simulink model "RealLifeTrainModel"  (R2024a)
settings: Solver=ode1  StartTime=0.0  StopTime=Inf  FixedStep=0.001  RelTol=1e-3
PostLoadFcn:
  | , if any(exist('dsrtsu_mdlpostloadfcn', 'file') ~= 0), dsrtsu_mdlpostloadfcn('Execute', bdroot); end,
InitFcn:
  | , if any(exist('rtifpga_mdlclblib', 'file') ~= 0), rtifpga_mdlclblib('Init', bdroot); end,
undefined symbols (not defined in the file): DiscIntNeverNeededParam
libraries: deeplib x29, svdutilitieslib x28, simulink x8, eeGeneralControl x8, rti1202lib_adc_class1 x6, rti1202serlib x5, spsEdgeDetectorLib x5, rtiemclib x2, rti1202lib_dac_class1 x1
(part 1 of 8)
Description:
  | Standard RTI1202 template.
  | Supported MATLAB version:  R2024a.
settings Model: Tag=RTI1202  DSRTSU_INTERNAL_RTI_VER=640  DSRTSU_INTERNAL_RTI_TYPE=rti1202  RTICANMMDATA=struct('GeneralSetupData',struct('modelroot','C:\Users\VM-User\Desktop\MigrationScripts','generalsettings',struct('filesettings',struct('destfolder',struct('Name','RTICANMM_FILES','Check',1),'buildfolder',struct('Name','.','Check',1),'AbsDestfolder',struct('Name','C:\Users\VM-User\Desktop\MigrationScripts\RTICANMM_FILES'),'AbsBuildfolder',struct('Name','C:\Users\VM-User\Desktop\MigrationScripts'))),'options',struct('addpaths',1,'rmpaths',1,'addtrcexclusion',true,'cannavigator',struct('checkmonitoring',0),'show_usrtrc',0,'use_usrtrc',0),'advanced',struct('options',ones(1,100)),'MPSetup',{{}},'RTI',struct('Type','RTI1202','Ver','7.17','Date','02-Nov-2021'),'modelname','','block','untitled'))  DSRTSU_INTERNAL_RTIFPGA=210  DSRTSU_INTERNAL_RTISTBM_VER=24.1  Creator=ic2d  LastModifiedBy=ic2d
settings SolverCC: AlgebraicLoopSolver=TrustRegion
settings DataIOCC: ReturnWorkspaceOutputs=off
settings OptimizationCC: BlockReduction=off  OptimizeBlockIOStorage=off  BufferReuse=off  ReuseModelBlockBuffer=off  GlobalBufferReuse=off  ExpressionFolding=off  LocalBlockOutputs=off  OptimizeDataStoreBuffers=off  BusAssignmentInplaceUpdate=off
settings DebuggingCC: MultiTaskDSMMsg=none  UnconnectedInputMsg=warning  UnconnectedOutputMsg=warning  UnconnectedLineMsg=warning  PregeneratedLibrarySubsystemCodeDiagnostic=none  ForceCombineOutputUpdateInSim=on  ArithmeticOperatorsInVariantConditions=warning
settings HardwareCC: ProdBitPerPointer=32  ProdBitPerSizeT=32  ProdBitPerPtrDiffT=32  ProdLargestAtomicInteger=Integer  ProdEndianess=BigEndian  ProdWordSize=32  ProdLongLongMode=on  ProdHWDeviceType=Custom Processor->Custom  TargetIntDivRoundTo=Zero  TargetEndianess=BigEndian  TargetHWDeviceType=Custom Processor->Custom
settings ModelReferenceCC: EnableRefExpFcnMdlSchedulingChecks=on  EnableParallelModelReferenceBuilds=on  ParallelModelReferenceMATLABWorkerInit=Load Top Model
settings SFSimCC: SimUseLocalCustomCode=off  MATLABDynamicMemAlloc=off  CustomCodeUndefinedFunction=UseInterfaceOnly
settings RTWCC: Description=dSPACE DS1202 Hardware Platform  SystemTargetFile=rti1202.tlc  MakeCommand=make_rti  TemplateMakefile=rti1202.tmf  RTWUseLocalCustomCode=off  GPUComputeCapability=3.5  DLArmComputeVersion=19.05
settings CodeAppCC: StateflowObjectComments=on
settings STFCustomTargetCC: TargetLangStandard=C89/C90 (ANSI)  ParMdlRefBuildCompliant=on  GRTInterface=off  UseToolchainInfoCompliant=off  SystemTargetFile=rti1202.tlc
settings GRTTargetCC: TargetLangStandard=C89/C90 (ANSI)  CompOptLevelCompliant=off  ConcurrentExecutionCompliant=off  CombineOutputUpdateFcns=off  MatFileLogging=off  CPPClassGenCompliant=off  UseToolchainInfoCompliant=off
settings ConfigComp: CovMetricSettings=dswe

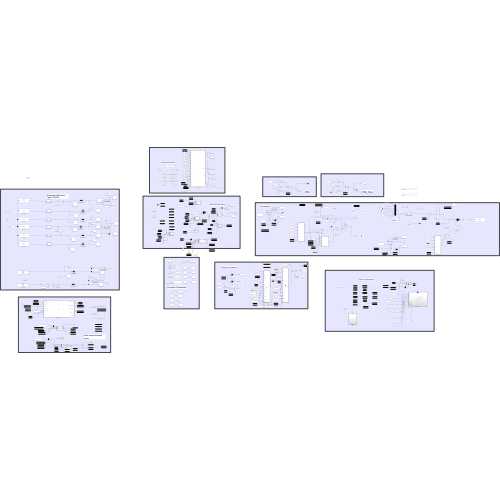
[thumbnail: Simulink's stored preview of the top-level diagram]
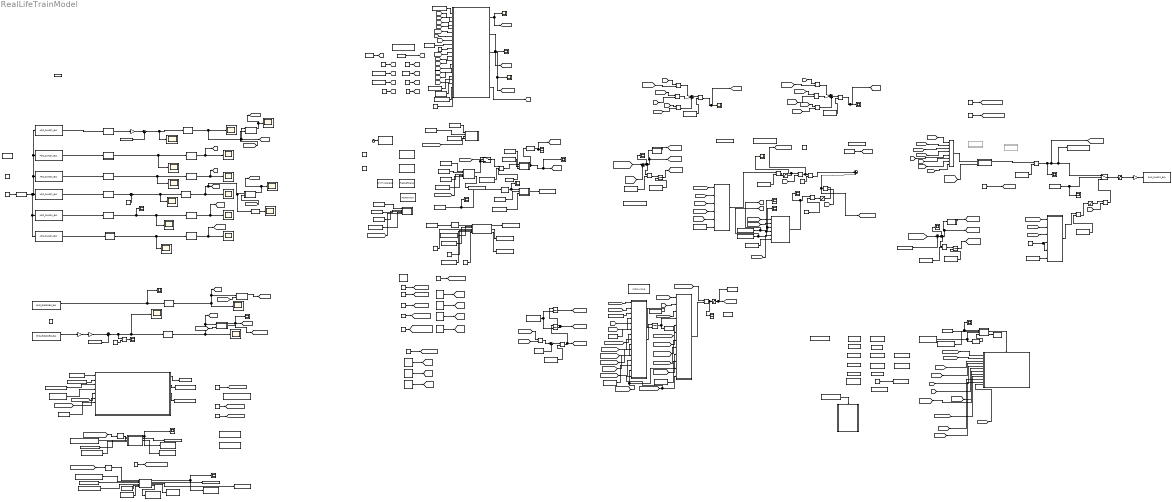
== system RealLifeTrainModel ==
  note: PID
  note: Start-Stop-Recording Logic
  note: Disturbance Estimation
  note: Controllers
  note: Hyd Model Parameters
  note: Controller Parameters
  note: Reference Generation
  note: Serial Communication
  note: Hardware Abstraction Layer (TODO)
  note: PID_Pos
  ADCReadToNewtons_Hyd : MATLAB Function  TreatAsAtomicUnit=on
  ADCReadToNewtons_Load : MATLAB Function  TreatAsAtomicUnit=on
  ADCReadToPressure : MATLAB Function  TreatAsAtomicUnit=on
  ADCReadToPressure1 : MATLAB Function  TreatAsAtomicUnit=on
  ADCReadToPressure2 : MATLAB Function  TreatAsAtomicUnit=on
  ADCReadToPressure3 : MATLAB Function  TreatAsAtomicUnit=on
  ADC_CLASS1_BL1 : rti1202lib_adc_class1/ADC_CLASS1_BL1  DSProperties=struct('RTI',struct('Version',uint32(1),'BlockType',struct('isSLSource',uint8(1),'isSLSink',uint8(1),'isHWSource',uint8(0),'isHWSink',uint8(1),'isSetup',uint8(0),'isInline',uint8(1),'isNonInline',uint8(0),'isInterrupt',uint8(0),'isChannelwise',uint8(1)),'IOBoardType',{{'DS120X','STD','ADCC1'}},'UnitType','ADC','Identifier','ADC','DialogType','ML','BlockSet','NONE','SlaveProcessor','NONE'))  RTIBlockInterface=struct('InputPortsActive',1,'InputPortsWidth',int32(1),'InputPortsDataType',{{'SS_BOOLEAN'}},'InputPortsName',{{'Continue'}},'OutputPortsActive',[1 0],'OutputPortsWidth',int32([100 1]),'OutputPortsDataType',{{'SS_DOUBLE','SS_INT16'}},'OutputPortsName',{{'ADC','Status'}},'DialogFcn','rti120xstdadcc1adcgui','SampleTime',{{-1}},'InitLevel',3,'IconTransparency','on','BlockDisplay',{{['ADC CL1\nChannel: 1'],'center'}},'BlockName',struct('Token',{{'ADC_CLASS1_BL1'}}))  RTIBlockParameters=struct('ReadMode',{{2,'OFF',[1 2]}},'ChannelNo',{{1,'OFF',[]}},'ConversionMode',{{2,'OFF',[1 2]}},'TriggerSource',{{1,'OFF',[1 2]}},'TriggerLineIn',{{1,'OFF',[1 16]}},'SampleMode',{{2,'OFF',[1 2]}},'BurstTriggerSource',{{1,'OFF',[1 2]}},'BurstTriggerLine',{{1,'OFF',[1 16]}},'ConvTriggerSource',{{3,'OFF',[1 3]}},'ConvTriggerLine',{{1,'OFF',[1 16]}},'ConvPeriod',{{'str2num(get_param(''Teste_PID/TimerValue'',''Value''))','OFF',[1e-6 1.34]}},'ConvPeriodCheck',{{1,'OFF',[]}},'BurstSize',{{'str2num(get_param(''Teste_PID/BufferSize'',''Value''))','OFF',[]}},'BurstSizeCheck',{{1,'OFF',[]}},'DataSetOffset',{{'0','OFF',[]}},'DataSetOffsetCheck',{{0,'OFF',[]}},'DataSetLength',{{'1','OFF',[]}},'DataSetLengthCheck',{{0,'OFF',[]}},'EnableTriggerEvent',{{0,'OFF',[0 1]}},'TriggerMode',{{2,'OFF',[1 3]}},'TriggerLineOut',{{1,'OFF',[1 16]}},'ADCSWStartEnable',{{0,'OFF',[0 1]}},'SampleTime',{{'-1','OFF',[-1 inf]}},'SampleTimeCheck',{{0,'OFF',[]}},'StatusPortEnable',{{0,'OFF',[0 1]}},'TLCFileName',{{'rti120xadc_c1_adc','OFF',[]}})  RTISFcnParameters=struct('ReadMode','int16','ChannelNo','int16','ConversionMode','int16','TriggerSource','int16','TriggerLineIn','int16','SampleMode','int16','BurstTriggerSource','int16','BurstTriggerLine','int16','ConvTriggerSource','int16','ConvTriggerLine','int16','ConvPeriod','double','BurstSize','int16','DataSetOffset','int16','DataSetLength','int16','EnableTriggerEvent','int16','TriggerMode','int16','TriggerLineOut','int16','ADCSWStartEnable','int16','SampleTime','double','StatusPortEnable','int16','TLCFileName','char')  RTIBlockParaDefault=struct('ReadMode',1,'ChannelNo',1,'ConversionMode',1,'TriggerSource',1,'TriggerLineIn',1,'SampleMode',1,'BurstTriggerSource',1,'BurstTriggerLine',1,'ConvTriggerSource',3,'ConvTriggerLine',1,'ConvPeriod',0.0001,'ConvPeriodCheck',0,'BurstSize',10,'BurstSizeCheck',0,'DataSetOffset',0,'DataSetOffsetCheck',0,'DataSetLength',1,'DataSetLengthCheck',0,'EnableTriggerEvent',0,'TriggerMode',2,'TriggerLineOut',1,'ADCSWStartEnable',0,'SampleTime',-1,'SampleTimeCheck',1,'StatusPortEnable',0,'TLCFileName','rti120xadc_c1_adc')
  ADC_CLASS1_BL2 : rti1202lib_adc_class1/ADC_CLASS1_BL1  DSProperties=struct('RTI',struct('Version',uint32(1),'BlockType',struct('isSLSource',uint8(1),'isSLSink',uint8(1),'isHWSource',uint8(0),'isHWSink',uint8(1),'isSetup',uint8(0),'isInline',uint8(1),'isNonInline',uint8(0),'isInterrupt',uint8(0),'isChannelwise',uint8(1)),'IOBoardType',{{'DS120X','STD','ADCC1'}},'UnitType','ADC','Identifier','ADC','DialogType','ML','BlockSet','NONE','SlaveProcessor','NONE'))  RTIBlockInterface=struct('InputPortsActive',1,'InputPortsWidth',int32(1),'InputPortsDataType',{{'SS_BOOLEAN'}},'InputPortsName',{{'Continue'}},'OutputPortsActive',[1 0],'OutputPortsWidth',int32([100 1]),'OutputPortsDataType',{{'SS_DOUBLE','SS_INT16'}},'OutputPortsName',{{'ADC','Status'}},'DialogFcn','rti120xstdadcc1adcgui','SampleTime',{{-1}},'InitLevel',3,'IconTransparency','on','BlockDisplay',{{['ADC CL1\nChannel: 13'],'center'}},'BlockName',struct('Token',{{'ADC_CLASS1_BL1'}}))  RTIBlockParameters=struct('ReadMode',{{2,'OFF',[1 2]}},'ChannelNo',{{13,'OFF',[]}},'ConversionMode',{{2,'OFF',[1 2]}},'TriggerSource',{{1,'OFF',[1 2]}},'TriggerLineIn',{{1,'OFF',[1 16]}},'SampleMode',{{2,'OFF',[1 2]}},'BurstTriggerSource',{{1,'OFF',[1 2]}},'BurstTriggerLine',{{1,'OFF',[1 16]}},'ConvTriggerSource',{{3,'OFF',[1 3]}},'ConvTriggerLine',{{1,'OFF',[1 16]}},'ConvPeriod',{{'str2num(get_param(''Teste_PID/TimerValue'',''Value''))','OFF',[1e-6 1.34]}},'ConvPeriodCheck',{{1,'OFF',[]}},'BurstSize',{{'str2num(get_param(''Teste_PID/BufferSize'',''Value''))','OFF',[]}},'BurstSizeCheck',{{1,'OFF',[]}},'DataSetOffset',{{'0','OFF',[]}},'DataSetOffsetCheck',{{0,'OFF',[]}},'DataSetLength',{{'1','OFF',[]}},'DataSetLengthCheck',{{0,'OFF',[]}},'EnableTriggerEvent',{{0,'OFF',[0 1]}},'TriggerMode',{{2,'OFF',[1 3]}},'TriggerLineOut',{{1,'OFF',[1 16]}},'ADCSWStartEnable',{{0,'OFF',[0 1]}},'SampleTime',{{'-1','OFF',[-1 inf]}},'SampleTimeCheck',{{0,'OFF',[]}},'StatusPortEnable',{{0,'OFF',[0 1]}},'TLCFileName',{{'rti120xadc_c1_adc','OFF',[]}})  RTISFcnParameters=struct('ReadMode','int16','ChannelNo','int16','ConversionMode','int16','TriggerSource','int16','TriggerLineIn','int16','SampleMode','int16','BurstTriggerSource','int16','BurstTriggerLine','int16','ConvTriggerSource','int16','ConvTriggerLine','int16','ConvPeriod','double','BurstSize','int16','DataSetOffset','int16','DataSetLength','int16','EnableTriggerEvent','int16','TriggerMode','int16','TriggerLineOut','int16','ADCSWStartEnable','int16','SampleTime','double','StatusPortEnable','int16','TLCFileName','char')  RTIBlockParaDefault=struct('ReadMode',1,'ChannelNo',1,'ConversionMode',1,'TriggerSource',1,'TriggerLineIn',1,'SampleMode',1,'BurstTriggerSource',1,'BurstTriggerLine',1,'ConvTriggerSource',3,'ConvTriggerLine',1,'ConvPeriod',0.0001,'ConvPeriodCheck',0,'BurstSize',10,'BurstSizeCheck',0,'DataSetOffset',0,'DataSetOffsetCheck',0,'DataSetLength',1,'DataSetLengthCheck',0,'EnableTriggerEvent',0,'TriggerMode',2,'TriggerLineOut',1,'ADCSWStartEnable',0,'SampleTime',-1,'SampleTimeCheck',1,'StatusPortEnable',0,'TLCFileName','rti120xadc_c1_adc')
  ADC_CLASS1_BL3 : rti1202lib_adc_class1/ADC_CLASS1_BL1  DSProperties=struct('RTI',struct('Version',uint32(1),'BlockType',struct('isSLSource',uint8(1),'isSLSink',uint8(1),'isHWSource',uint8(0),'isHWSink',uint8(1),'isSetup',uint8(0),'isInline',uint8(1),'isNonInline',uint8(0),'isInterrupt',uint8(0),'isChannelwise',uint8(1)),'IOBoardType',{{'DS120X','STD','ADCC1'}},'UnitType','ADC','Identifier','ADC','DialogType','ML','BlockSet','NONE','SlaveProcessor','NONE'))  RTIBlockInterface=struct('InputPortsActive',1,'InputPortsWidth',int32(1),'InputPortsDataType',{{'SS_BOOLEAN'}},'InputPortsName',{{'Continue'}},'OutputPortsActive',[1 0],'OutputPortsWidth',int32([100 1]),'OutputPortsDataType',{{'SS_DOUBLE','SS_INT16'}},'OutputPortsName',{{'ADC','Status'}},'DialogFcn','rti120xstdadcc1adcgui','SampleTime',{{-1}},'InitLevel',3,'IconTransparency','on','BlockDisplay',{{['ADC CL1\nChannel: 5'],'center'}},'BlockName',struct('Token',{{'ADC_CLASS1_BL1'}}))  RTIBlockParameters=struct('ReadMode',{{2,'OFF',[1 2]}},'ChannelNo',{{5,'OFF',[]}},'ConversionMode',{{2,'OFF',[1 2]}},'TriggerSource',{{1,'OFF',[1 2]}},'TriggerLineIn',{{1,'OFF',[1 16]}},'SampleMode',{{2,'OFF',[1 2]}},'BurstTriggerSource',{{1,'OFF',[1 2]}},'BurstTriggerLine',{{1,'OFF',[1 16]}},'ConvTriggerSource',{{3,'OFF',[1 3]}},'ConvTriggerLine',{{1,'OFF',[1 16]}},'ConvPeriod',{{'str2num(get_param(''Teste_PID/TimerValue'',''Value''))','OFF',[1e-6 1.34]}},'ConvPeriodCheck',{{1,'OFF',[]}},'BurstSize',{{'str2num(get_param(''Teste_PID/BufferSize'',''Value''))','OFF',[]}},'BurstSizeCheck',{{1,'OFF',[]}},'DataSetOffset',{{'0','OFF',[]}},'DataSetOffsetCheck',{{0,'OFF',[]}},'DataSetLength',{{'1','OFF',[]}},'DataSetLengthCheck',{{0,'OFF',[]}},'EnableTriggerEvent',{{0,'OFF',[0 1]}},'TriggerMode',{{2,'OFF',[1 3]}},'TriggerLineOut',{{1,'OFF',[1 16]}},'ADCSWStartEnable',{{0,'OFF',[0 1]}},'SampleTime',{{'-1','OFF',[-1 inf]}},'SampleTimeCheck',{{0,'OFF',[]}},'StatusPortEnable',{{0,'OFF',[0 1]}},'TLCFileName',{{'rti120xadc_c1_adc','OFF',[]}})  RTISFcnParameters=struct('ReadMode','int16','ChannelNo','int16','ConversionMode','int16','TriggerSource','int16','TriggerLineIn','int16','SampleMode','int16','BurstTriggerSource','int16','BurstTriggerLine','int16','ConvTriggerSource','int16','ConvTriggerLine','int16','ConvPeriod','double','BurstSize','int16','DataSetOffset','int16','DataSetLength','int16','EnableTriggerEvent','int16','TriggerMode','int16','TriggerLineOut','int16','ADCSWStartEnable','int16','SampleTime','double','StatusPortEnable','int16','TLCFileName','char')  RTIBlockParaDefault=struct('ReadMode',1,'ChannelNo',1,'ConversionMode',1,'TriggerSource',1,'TriggerLineIn',1,'SampleMode',1,'BurstTriggerSource',1,'BurstTriggerLine',1,'ConvTriggerSource',3,'ConvTriggerLine',1,'ConvPeriod',0.0001,'ConvPeriodCheck',0,'BurstSize',10,'BurstSizeCheck',0,'DataSetOffset',0,'DataSetOffsetCheck',0,'DataSetLength',1,'DataSetLengthCheck',0,'EnableTriggerEvent',0,'TriggerMode',2,'TriggerLineOut',1,'ADCSWStartEnable',0,'SampleTime',-1,'SampleTimeCheck',1,'StatusPortEnable',0,'TLCFileName','rti120xadc_c1_adc')
  ADC_CLASS1_BL4 : rti1202lib_adc_class1/ADC_CLASS1_BL1  DSProperties=struct('RTI',struct('Version',uint32(1),'BlockType',struct('isSLSource',uint8(1),'isSLSink',uint8(1),'isHWSource',uint8(0),'isHWSink',uint8(1),'isSetup',uint8(0),'isInline',uint8(1),'isNonInline',uint8(0),'isInterrupt',uint8(0),'isChannelwise',uint8(1)),'IOBoardType',{{'DS120X','STD','ADCC1'}},'UnitType','ADC','Identifier','ADC','DialogType','ML','BlockSet','NONE','SlaveProcessor','NONE'))  RTIBlockInterface=struct('InputPortsActive',1,'InputPortsWidth',int32(1),'InputPortsDataType',{{'SS_BOOLEAN'}},'InputPortsName',{{'Continue'}},'OutputPortsActive',[1 0],'OutputPortsWidth',int32([100 1]),'OutputPortsDataType',{{'SS_DOUBLE','SS_INT16'}},'OutputPortsName',{{'ADC','Status'}},'DialogFcn','rti120xstdadcc1adcgui','SampleTime',{{-1}},'InitLevel',3,'IconTransparency','on','BlockDisplay',{{['ADC CL1\nChannel: 2'],'center'}},'BlockName',struct('Token',{{'ADC_CLASS1_BL1'}}))  RTIBlockParameters=struct('ReadMode',{{2,'OFF',[1 2]}},'ChannelNo',{{2,'OFF',[]}},'ConversionMode',{{2,'OFF',[1 2]}},'TriggerSource',{{1,'OFF',[1 2]}},'TriggerLineIn',{{1,'OFF',[1 16]}},'SampleMode',{{2,'OFF',[1 2]}},'BurstTriggerSource',{{1,'OFF',[1 2]}},'BurstTriggerLine',{{1,'OFF',[1 16]}},'ConvTriggerSource',{{3,'OFF',[1 3]}},'ConvTriggerLine',{{1,'OFF',[1 16]}},'ConvPeriod',{{'str2num(get_param(''Teste_PID/TimerValue'',''Value''))','OFF',[1e-6 1.34]}},'ConvPeriodCheck',{{1,'OFF',[]}},'BurstSize',{{'str2num(get_param(''Teste_PID/BufferSize'',''Value''))','OFF',[]}},'BurstSizeCheck',{{1,'OFF',[]}},'DataSetOffset',{{'0','OFF',[]}},'DataSetOffsetCheck',{{0,'OFF',[]}},'DataSetLength',{{'1','OFF',[]}},'DataSetLengthCheck',{{0,'OFF',[]}},'EnableTriggerEvent',{{0,'OFF',[0 1]}},'TriggerMode',{{2,'OFF',[1 3]}},'TriggerLineOut',{{1,'OFF',[1 16]}},'ADCSWStartEnable',{{0,'OFF',[0 1]}},'SampleTime',{{'-1','OFF',[-1 inf]}},'SampleTimeCheck',{{0,'OFF',[]}},'StatusPortEnable',{{0,'OFF',[0 1]}},'TLCFileName',{{'rti120xadc_c1_adc','OFF',[]}})  RTISFcnParameters=struct('ReadMode','int16','ChannelNo','int16','ConversionMode','int16','TriggerSource','int16','TriggerLineIn','int16','SampleMode','int16','BurstTriggerSource','int16','BurstTriggerLine','int16','ConvTriggerSource','int16','ConvTriggerLine','int16','ConvPeriod','double','BurstSize','int16','DataSetOffset','int16','DataSetLength','int16','EnableTriggerEvent','int16','TriggerMode','int16','TriggerLineOut','int16','ADCSWStartEnable','int16','SampleTime','double','StatusPortEnable','int16','TLCFileName','char')  RTIBlockParaDefault=struct('ReadMode',1,'ChannelNo',1,'ConversionMode',1,'TriggerSource',1,'TriggerLineIn',1,'SampleMode',1,'BurstTriggerSource',1,'BurstTriggerLine',1,'ConvTriggerSource',3,'ConvTriggerLine',1,'ConvPeriod',0.0001,'ConvPeriodCheck',0,'BurstSize',10,'BurstSizeCheck',0,'DataSetOffset',0,'DataSetOffsetCheck',0,'DataSetLength',1,'DataSetLengthCheck',0,'EnableTriggerEvent',0,'TriggerMode',2,'TriggerLineOut',1,'ADCSWStartEnable',0,'SampleTime',-1,'SampleTimeCheck',1,'StatusPortEnable',0,'TLCFileName','rti120xadc_c1_adc')
  ADC_CLASS1_BL5 : rti1202lib_adc_class1/ADC_CLASS1_BL1  DSProperties=struct('RTI',struct('Version',uint32(1),'BlockType',struct('isSLSource',uint8(1),'isSLSink',uint8(1),'isHWSource',uint8(0),'isHWSink',uint8(1),'isSetup',uint8(0),'isInline',uint8(1),'isNonInline',uint8(0),'isInterrupt',uint8(0),'isChannelwise',uint8(1)),'IOBoardType',{{'DS120X','STD','ADCC1'}},'UnitType','ADC','Identifier','ADC','DialogType','ML','BlockSet','NONE','SlaveProcessor','NONE'))  RTIBlockInterface=struct('InputPortsActive',1,'InputPortsWidth',int32(1),'InputPortsDataType',{{'SS_BOOLEAN'}},'InputPortsName',{{'Continue'}},'OutputPortsActive',[1 0],'OutputPortsWidth',int32([100 1]),'OutputPortsDataType',{{'SS_DOUBLE','SS_INT16'}},'OutputPortsName',{{'ADC','Status'}},'DialogFcn','rti120xstdadcc1adcgui','SampleTime',{{-1}},'InitLevel',3,'IconTransparency','on','BlockDisplay',{{['ADC CL1\nChannel: 15'],'center'}},'BlockName',struct('Token',{{'ADC_CLASS1_BL1'}}))  RTIBlockParameters=struct('ReadMode',{{2,'OFF',[1 2]}},'ChannelNo',{{15,'OFF',[]}},'ConversionMode',{{2,'OFF',[1 2]}},'TriggerSource',{{1,'OFF',[1 2]}},'TriggerLineIn',{{1,'OFF',[1 16]}},'SampleMode',{{2,'OFF',[1 2]}},'BurstTriggerSource',{{1,'OFF',[1 2]}},'BurstTriggerLine',{{1,'OFF',[1 16]}},'ConvTriggerSource',{{3,'OFF',[1 3]}},'ConvTriggerLine',{{1,'OFF',[1 16]}},'ConvPeriod',{{'str2num(get_param(''Teste_PID/TimerValue'',''Value''))','OFF',[1e-6 1.34]}},'ConvPeriodCheck',{{1,'OFF',[]}},'BurstSize',{{'str2num(get_param(''Teste_PID/BufferSize'',''Value''))','OFF',[]}},'BurstSizeCheck',{{1,'OFF',[]}},'DataSetOffset',{{'0','OFF',[]}},'DataSetOffsetCheck',{{0,'OFF',[]}},'DataSetLength',{{'1','OFF',[]}},'DataSetLengthCheck',{{0,'OFF',[]}},'EnableTriggerEvent',{{0,'OFF',[0 1]}},'TriggerMode',{{2,'OFF',[1 3]}},'TriggerLineOut',{{1,'OFF',[1 16]}},'ADCSWStartEnable',{{0,'OFF',[0 1]}},'SampleTime',{{'-1','OFF',[-1 inf]}},'SampleTimeCheck',{{0,'OFF',[]}},'StatusPortEnable',{{0,'OFF',[0 1]}},'TLCFileName',{{'rti120xadc_c1_adc','OFF',[]}})  RTISFcnParameters=struct('ReadMode','int16','ChannelNo','int16','ConversionMode','int16','TriggerSource','int16','TriggerLineIn','int16','SampleMode','int16','BurstTriggerSource','int16','BurstTriggerLine','int16','ConvTriggerSource','int16','ConvTriggerLine','int16','ConvPeriod','double','BurstSize','int16','DataSetOffset','int16','DataSetLength','int16','EnableTriggerEvent','int16','TriggerMode','int16','TriggerLineOut','int16','ADCSWStartEnable','int16','SampleTime','double','StatusPortEnable','int16','TLCFileName','char')  RTIBlockParaDefault=struct('ReadMode',1,'ChannelNo',1,'ConversionMode',1,'TriggerSource',1,'TriggerLineIn',1,'SampleMode',1,'BurstTriggerSource',1,'BurstTriggerLine',1,'ConvTriggerSource',3,'ConvTriggerLine',1,'ConvPeriod',0.0001,'ConvPeriodCheck',0,'BurstSize',10,'BurstSizeCheck',0,'DataSetOffset',0,'DataSetOffsetCheck',0,'DataSetLength',1,'DataSetLengthCheck',0,'EnableTriggerEvent',0,'TriggerMode',2,'TriggerLineOut',1,'ADCSWStartEnable',0,'SampleTime',-1,'SampleTimeCheck',1,'StatusPortEnable',0,'TLCFileName','rti120xadc_c1_adc')
  ADC_CLASS1_BL6 : rti1202lib_adc_class1/ADC_CLASS1_BL1  DSProperties=struct('RTI',struct('Version',uint32(1),'BlockType',struct('isSLSource',uint8(1),'isSLSink',uint8(1),'isHWSource',uint8(0),'isHWSink',uint8(1),'isSetup',uint8(0),'isInline',uint8(1),'isNonInline',uint8(0),'isInterrupt',uint8(0),'isChannelwise',uint8(1)),'IOBoardType',{{'DS120X','STD','ADCC1'}},'UnitType','ADC','Identifier','ADC','DialogType','ML','BlockSet','NONE','SlaveProcessor','NONE'))  RTIBlockInterface=struct('InputPortsActive',1,'InputPortsWidth',int32(1),'InputPortsDataType',{{'SS_BOOLEAN'}},'InputPortsName',{{'Continue'}},'OutputPortsActive',[1 0],'OutputPortsWidth',int32([100 1]),'OutputPortsDataType',{{'SS_DOUBLE','SS_INT16'}},'OutputPortsName',{{'ADC','Status'}},'DialogFcn','rti120xstdadcc1adcgui','SampleTime',{{-1}},'InitLevel',3,'IconTransparency','on','BlockDisplay',{{['ADC CL1\nChannel: 7'],'center'}},'BlockName',struct('Token',{{'ADC_CLASS1_BL1'}}))  RTIBlockParameters=struct('ReadMode',{{2,'OFF',[1 2]}},'ChannelNo',{{7,'OFF',[]}},'ConversionMode',{{2,'OFF',[1 2]}},'TriggerSource',{{1,'OFF',[1 2]}},'TriggerLineIn',{{1,'OFF',[1 16]}},'SampleMode',{{2,'OFF',[1 2]}},'BurstTriggerSource',{{1,'OFF',[1 2]}},'BurstTriggerLine',{{1,'OFF',[1 16]}},'ConvTriggerSource',{{3,'OFF',[1 3]}},'ConvTriggerLine',{{1,'OFF',[1 16]}},'ConvPeriod',{{'str2num(get_param(''Teste_PID/TimerValue'',''Value''))','OFF',[1e-6 1.34]}},'ConvPeriodCheck',{{1,'OFF',[]}},'BurstSize',{{'str2num(get_param(''Teste_PID/BufferSize'',''Value''))','OFF',[]}},'BurstSizeCheck',{{1,'OFF',[]}},'DataSetOffset',{{'0','OFF',[]}},'DataSetOffsetCheck',{{0,'OFF',[]}},'DataSetLength',{{'1','OFF',[]}},'DataSetLengthCheck',{{0,'OFF',[]}},'EnableTriggerEvent',{{0,'OFF',[0 1]}},'TriggerMode',{{2,'OFF',[1 3]}},'TriggerLineOut',{{1,'OFF',[1 16]}},'ADCSWStartEnable',{{0,'OFF',[0 1]}},'SampleTime',{{'-1','OFF',[-1 inf]}},'SampleTimeCheck',{{0,'OFF',[]}},'StatusPortEnable',{{0,'OFF',[0 1]}},'TLCFileName',{{'rti120xadc_c1_adc','OFF',[]}})  RTISFcnParameters=struct('ReadMode','int16','ChannelNo','int16','ConversionMode','int16','TriggerSource','int16','TriggerLineIn','int16','SampleMode','int16','BurstTriggerSource','int16','BurstTriggerLine','int16','ConvTriggerSource','int16','ConvTriggerLine','int16','ConvPeriod','double','BurstSize','int16','DataSetOffset','int16','DataSetLength','int16','EnableTriggerEvent','int16','TriggerMode','int16','TriggerLineOut','int16','ADCSWStartEnable','int16','SampleTime','double','StatusPortEnable','int16','TLCFileName','char')  RTIBlockParaDefault=struct('ReadMode',1,'ChannelNo',1,'ConversionMode',1,'TriggerSource',1,'TriggerLineIn',1,'SampleMode',1,'BurstTriggerSource',1,'BurstTriggerLine',1,'ConvTriggerSource',3,'ConvTriggerLine',1,'ConvPeriod',0.0001,'ConvPeriodCheck',0,'BurstSize',10,'BurstSizeCheck',0,'DataSetOffset',0,'DataSetOffsetCheck',0,'DataSetLength',1,'DataSetLengthCheck',0,'EnableTriggerEvent',0,'TriggerMode',2,'TriggerLineOut',1,'ADCSWStartEnable',0,'SampleTime',-1,'SampleTimeCheck',1,'StatusPortEnable',0,'TLCFileName','rti120xadc_c1_adc')
  AmplitureRefSignaValue : Constant  Value=300
  AmplitureRefSignalMemory : DataStoreMemory  DataStoreName=AmplitureRefSignal  WriteAfterWriteMsg=warning  ShowAdditionalParam=off
  AmplitureRefSignalRead : DataStoreRead  DataStoreName=AmplitureRefSignal  IndexOptions=Index vector (dialog)  Indices=1  OutputSizes=1
  AmplitureRefSignalRead1 : DataStoreRead  DataStoreName=AmplitureRefSignal  IndexOptions=Index vector (dialog)  Indices=1  OutputSizes=1
  AmplitureRefSignalRead2 : DataStoreRead  DataStoreName=AmplitureRefSignal  IndexOptions=Index vector (dialog)  Indices=1  OutputSizes=1
  BufferSize : Constant  Value=100
  Bulk : Constant  Value=1.31E+9
  C1 : Constant  Value=0.8
  C2 : Constant
  Cast To Boolean : DataTypeConversion  OutDataTypeStr=boolean  SaturateOnIntegerOverflow=off  RndMeth=Floor
  Cli : Constant  Value=4e-13
  Clock : Clock
  CommSystem : Subsystem  TreatAsAtomicUnit=on
  Constant : Constant  Value=0
  Constant1 : Constant  Value=20000
  Constant2 : Constant  Value=10
  Constant4 : Constant
  Constant5 : Constant  Value=20
  Constant6 : Constant  Value=16000000
  Constant7 : Constant  Value=0
  ContractionMetricFilterSystem1 : Subsystem
  ContractionMetricFilterSystem2 : Subsystem  Commented=on
  ContractionMetricFilterSystem3 : Subsystem  Commented=on
  ControlGain : Constant
  CylinderArea : Constant  Value=0.000201
  CylinderAreaRatio : Constant  Value=0.609
  DAC_CLASS1_BL1 : rti1202lib_dac_class1/DAC_CLASS1_BL1  DSProperties=struct('RTI',struct('Version',uint32(2),'BlockType',struct('isSLSource',uint8(0),'isSLSink',uint8(1),'isHWSource',uint8(0),'isHWSink',uint8(1),'isSetup',uint8(0),'isInline',uint8(1),'isNonInline',uint8(0),'isInterrupt',uint8(0),'isChannelwise',uint8(1)),'IOBoardType',{{'DS120X','STD','DACC1'}},'UnitType','DAC','Identifier','DAC','DialogType','ML','BlockSet','NONE','SlaveProcessor','NONE'))  RTIBlockInterface=struct('InputPortsActive',1,'InputPortsWidth',int32(1),'InputPortsDataType',{{'SS_DOUBLE'}},'InputPortsName',{{['DAC 8']}},'DialogFcn','rti120xstddacc1dacgui','InitLevel',3,'IconTransparency','on','BlockDisplay',{{['DAC CL1\nChannel: 8'],'center'}},'BlockName',struct('Token',{{'DAC_CLASS1_BL1'}}))  RTIBlockParameters=struct('ChannelNo',{{8,'OFF',[]}},'ChannelNumOf',{{1,'OFF',[]}},'InitialValue1',{{'0','OFF',[-10 10]}},'InitialValue2',{{'0','OFF',[-10 10]}},'InitialValue3',{{'0','OFF',[-10 10]}},'InitialValue4',{{'0','OFF',[-10 10]}},'InitialValue5',{{'0','OFF',[-10 10]}},'InitialValue6',{{'0','OFF',[-10 10]}},'InitialValue7',{{'0','OFF',[-10 10]}},'InitialValue8',{{'0','OFF',[-10 10]}},'InitialValue9',{{'0','OFF',[-10 10]}},'InitialValue10',{{'0','OFF',[-10 10]}},'InitialValue11',{{'0','OFF',[-10 10]}},'InitialValue12',{{'0','OFF',[-10 10]}},'InitialValue13',{{'0','OFF',[-10 10]}},'InitialValue14',{{'0','OFF',[-10 10]}},'InitialValue15',{{'0','OFF',[-10 10]}},'InitialValue16',{{'0','OFF',[-10 10]}},'OutputMode',{{ones(1,16),'OFF',[1 2]}},'TermValue1',{{'0','OFF',[-10 10]}},'TermValue2',{{'0','OFF',[-10 10]}},'TermValue3',{{'0','OFF',[-10 10]}},'TermValue4',{{'0','OFF',[-10 10]}},'TermValue5',{{'0','OFF',[-10 10]}},'TermValue6',{{'0','OFF',[-10 10]}},'TermValue7',{{'0','OFF',[-10 10]}},'TermValue8',{{'0','OFF',[-10 10]}},'TermValue9',{{'0','OFF',[-10 10]}},'TermValue10',{{'0','OFF',[-10 10]}},'TermValue11',{{'0','OFF',[-10 10]}},'TermValue12',{{'0','OFF',[-10 10]}},'TermValue13',{{'0','OFF',[-10 10]}},'TermValue14',{{'0','OFF',[-10 10]}},'TermValue15',{{'0','OFF',[-10 10]}},'TermValue16',{{'0','OFF',[-10 10]}},'EnableTermMode',{{0,'OFF',[0 1]}},'TLCFileName',{{'rti120xdac_c1_dac','OFF',[]}},'InitialValueBuildCheck1',{{0,'OFF',[]}},'InitialValueBuildCheck2',{{0,'OFF',[]}},'InitialValueBuildCheck3',{{0,'OFF',[]}},'InitialValueBuildCheck4',{{0,'OFF',[]}},'InitialValueBuildCheck5',{{0,'OFF',[]}},'InitialValueBuildCheck6',{{0,'OFF',[]}},'InitialValueBuildCheck7',{{0,'OFF',[]}},'InitialValueBuildCheck8',{{1,'OFF',[]}},'InitialValueBuildCheck9',{{0,'OFF',[]}},'InitialValueBuildCheck10',{{0,'OFF',[]}},'InitialValueBuildCheck11',{{0,'OFF',[]}},'InitialValueBuildCheck12',{{0,'OFF',[]}},'InitialValueBuildCheck13',{{0,'OFF',[]}},'InitialValueBuildCheck14',{{0,'OFF',[]}},'InitialValueBuildCheck15',{{0,'OFF',[]}},'InitialValueBuildCheck16',{{0,'OFF',[]}},'TermValueBuildCheck1',{{0,'OFF',[]}},'TermValueBuildCheck2',{{0,'OFF',[]}},'TermValueBuildCheck3',{{0,'OFF',[]}},'TermValueBuildCheck4',{{0,'OFF',[]}},'TermValueBuildCheck5',{{0,'OFF',[]}},'TermValueBuildCheck6',{{0,'OFF',[]}},'TermValueBuildCheck7',{{0,'OFF',[]}},'TermValueBuildCheck8',{{0,'OFF',[]}},'TermValueBuildCheck9',{{0,'OFF',[]}},'TermValueBuildCheck10',{{0,'OFF',[]}},'TermValueBuildCheck11',{{0,'OFF',[]}},'TermValueBuildCheck12',{{0,'OFF',[]}},'TermValueBuildCheck13',{{0,'OFF',[]}},'TermValueBuildCheck14',{{0,'OFF',[]}},'TermValueBuildCheck15',{{0,'OFF',[]}},'TermValueBuildCheck16',{{0,'OFF',[]}})  RTISFcnParameters=struct('ChannelNo','int16','ChannelNumOf','int16','InitialValue1','double','InitialValue2','double','InitialValue3','double','InitialValue4','double','InitialValue5','double','InitialValue6','double','InitialValue7','double','InitialValue8','double','InitialValue9','double','InitialValue10','double','InitialValue11','double','InitialValue12','double','InitialValue13','double','InitialValue14','double','InitialValue15','double','InitialValue16','double','OutputMode','int16','TermValue1','double','TermValue2','double','TermValue3','double','TermValue4','double','TermValue5','double','TermValue6','double','TermValue7','double','TermValue8','double','TermValue9','double','TermValue10','double','TermValue11','double','TermValue12','double','TermValue13','double','TermValue14','double','TermValue15','double','TermValue16','double','EnableTermMode','int16','TLCFileName','char')  RTIBlockParaDefault=struct('ChannelNo',1,'ChannelNumOf',1,'InitialValue1',0,'InitialValue2',0,'InitialValue3',0,'InitialValue4',0,'InitialValue5',0,'InitialValue6',0,'InitialValue7',0,'InitialValue8',0,'InitialValue9',0,'InitialValue10',0,'InitialValue11',0,'InitialValue12',0,'InitialValue13',0,'InitialValue14',0,'InitialValue15',0,'InitialValue16',0,'OutputMode',ones(1,16),'TermValue1',0,'TermValue2',0,'TermValue3',0,'TermValue4',0,'TermValue5',0,'TermValue6',0,'TermValue7',0,'TermValue8',0,'TermValue9',0,'TermValue10',0,'TermValue11',0,'TermValue12',0,'TermValue13',0,'TermValue14',0,'TermValue15',0,'TermValue16',0,'EnableTermMode',0,'TLCFileName','rti120xdac_c1_dac','InitialValueBuildCheck1',0,'InitialValueBuildCheck2',0,'InitialValueBuildCheck3',0,'InitialValueBuildCheck4',0,'InitialValueBuildCheck5',0,'InitialValueBuildCheck6',0,'InitialValueBuildCheck7',0,'InitialValueBuildCheck8',0,'InitialValueBuildCheck9',0,'InitialValueBuildCheck10',0,'InitialValueBuildCheck11',0,'InitialValueBuildCheck12',0,'InitialValueBuildCheck13',0,'InitialValueBuildCheck14',0,'InitialValueBuildCheck15',0,'InitialValueBuildCheck16',0,'TermValueBuildCheck1',0,'TermValueBuildCheck2',0,'TermValueBuildCheck3',0,'TermValueBuildCheck4',0,'TermValueBuildCheck5',0,'TermValueBuildCheck6',0,'TermValueBuildCheck7',0,'TermValueBuildCheck8',0,'TermValueBuildCheck9',0,'TermValueBuildCheck10',0,'TermValueBuildCheck11',0,'TermValueBuildCheck12',0,'TermValueBuildCheck13',0,'TermValueBuildCheck14',0,'TermValueBuildCheck15',0,'TermValueBuildCheck16',0)
  DOBSat : Constant  Value=0.0001
  DS1202SER_INT_C1_I1 : rti1202serlib/DS1202SER_INT_C1_I1  Reserved1=[]  Reserved2=[]  Reserved3=[]  Reserved4=[]  DSProperties=struct('RTI',struct('IOBoardType',{{'DS1202','SER'}},'Version',uint32(530),'SlaveProcessor','NONE','BlockType',struct('isSLSource',uint8(1),'isSLSink',uint8(0),'isHWSource',uint8(0),'isHWSink',uint8(0),'isSetup',uint8(0),'isInline',uint8(1),'isNonInline',uint8(0),'isInterrupt',uint8(1),'isChannelwise',uint8(1)),'UnitType','GENSER','Identifier','SERINT','DialogType','ML','BlockSet','NONE','RelationId',struct('TH',struct('BlockId','HWINT'))))  RTIBlockInterface=struct('BlockDisplay',{{['DS1202 SER Interrupt\n Channel 1\nReceive Interrupt'],'center'}},'BlockName',struct('Token',{{'DS1202SER_INT_C','_I'}},'BlockParam',{{'ChannelNo','IntType'}}),'OutputPortsWidth',int32(1),'OutputPortsActive',1,'OutputPortsName',{{[' ']}},'IconTransparency','off','ParameterTunableNames',{{}},'InitLevel',3,'DialogFcn','guigenserserint','MaskDescription',['To make the interrupts of the UART serial interface available as trigger source.'],'FunctionCall',uint32(0),'Options',{{'SS_OPTION_FORCE_NONINLINED_FCNCALL','SS_OPTION_ASYNCHRONOUS_INTERRUPT'}},'OutputPortsDataType',{{'SS_FCN_CALL'}})  RTIBlockParameters=struct('ThIntNo',{{'UART_EVENTS','OFF',[]}},'ThSubIntNo',{{0,'ON',[0 4]}},'ThSrcSgnName',{{['UART Ch1 RX SW FIFO interrupt'],'OFF',[]}},'TLCFileName',{{'rti_hwinterrupt','OFF',[]}},'BoardNo',{{1,'ON',[1 1]}},'ChannelNo',{{1,'ON',[1 2]}},'ChannelNumOf',{{2,'OFF',[]}},'ThBlk',{{['struct(''blkh'',''Teste_PID/DS1202SER_INT_C1_I1'',''srcId'',''UART_EVENTS_CH1_INT0'',''srcSgnId'',''UART_EVENTS_CH1_INT0'',''intervalTmrBlockId'',[],''srcSgnName'',[''UART Ch1 RX SW FIFO interrupt''],''srcCpuId'','''',''isSrcCpu'',1,''isTargetCpu'',1,''srcOnMasterCpu'',1,''boardType'','''',''boardTypeNo'','''',''boardNo'',1,''intNo'',''UART_EVENTS'',''subIntNo'',0,''period'',0,''entryPoint'',''rti_UART_EVENTS_CH1_INT0'',''blockName'',''DS1202SER_INT_C1_I1'',''taskNameDisplayExt'','''',''taskType'',''HWINT'',''groupId'',''SERINT'',''hookFcn'',''NULL'',''isTimerTaskSrc'',0,''service'','''',''mpBlkId'','''',''taskPriorityPreConfig'',''none'',''taskPriority'',-1,''taskSortWeighting'',[],''taskSchedulingPolicy'',''FCFS'',''taskOvrPreConfig'',''none'',''taskOvrStrategy'',1,''taskOvrQueueSize'',1,''taskVisibility'',''on'',''taskGroupId'','''',''taskGroupDisplayOrder'',[],''serviceDynamicGen'',0,''disableCodeGen'',0,''boardBase'',''IOLIB_SPEC_INT_UART(1)'',''noBoardBase'','''')'],'OFF',[]}},'IntType',{{1,'ON',[1 4]}},'ReceiveIntLevelFifo',{{'7','OFF',[]}},'IntTypeMacro',{{'DSSER_TRIGGER_LEVEL_SUBINT_MASK','OFF',[]}},'FifoSizeDefault',{{64,'OFF',[]}})  RTISFcnParameters=struct('BoardNo','double','ChannelNo','double','ThIntNo','double','ThSubIntNo','double','ThBlk','struct','IntType','double','ReceiveIntLevelFifo','double','TLCFileName','char','IntTypeMacro','char')  RTIBlockParaDefault=struct('ThIntNo',1,'ThSubIntNo',0,'ThSrcSgnName',['RX SW FIFO interrupt'],'TLCFileName','rti_hwinterrupt','BoardNo',1,'ChannelNo',1,'ChannelNumOf',2,'ThBlk',['struct(''srcSgnId'', '''')'],'IntType',1,'ReceiveIntLevelFifo',1,'IntTypeMacro','DSSER_TRIGGER_LEVEL_SUBINT_MASK','FifoSizeDefault',64)
  DS1202SER_SETUP_C1 : rti1202serlib/DS1202SER_SETUP_C1  Reserved1=[]  Reserved2=[]  Reserved3=[]  Reserved4=[]  DSProperties=struct('RTI',struct('Version',uint32(2),'IOBoardType',{{'DS1202','SER'}},'SlaveProcessor','NONE','BlockType',struct('isSLSource',uint8(0),'isSLSink',uint8(0),'isHWSource',uint8(0),'isHWSink',uint8(0),'isSetup',uint8(1),'isInline',uint8(1),'isNonInline',uint8(0),'isInterrupt',uint8(0),'isChannelwise',uint8(1)),'UnitType','GENSER','Identifier','SETUP','DialogType','ML','BlockSet','NONE'))  RTIBlockInterface=struct('BlockName',struct('Token',{{'DS1202SER_SETUP_C'}},'BlockParam',{{'ChannelNo'}}),'BlockDisplay',{{['Serial Setup'],'center'}},'IconTransparency','off','ParameterTunableNames',{{}},'InitLevel',1,'DialogFcn','guigensersetup','MaskDescription',['To set the global specifications for the UART interface.'])  RTIBlockParameters=struct('ParityMode',{{1,'OFF',[1 5]}},'TransceiverMode',{{[1;1],'OFF',[]}},'QuartzFrequency',{{'160000000','OFF',[]}},'BoardNo',{{1,'ON',[1 1]}},'ChannelNo',{{1,'ON',[1 2]}},'ChannelNumOf',{{2,'OFF',[]}},'BaudRate',{{'230400','OFF',[]}},'DataBitsNumOf',{{4,'OFF',[1 4]}},'StopBitsNumOf',{{1,'OFF',[1 3]}},'ReceiveIntLevelUart',{{1,'OFF',[1 4]}},'AutoflowMode',{{0,'OFF',[]}},'FifoSize',{{'4096','OFF',[]}},'ReceiveIntLevelFifo',{{0,'OFF',[]}},'FifoOverrunMode',{{1,'OFF',[]}},'FifoBlockSize',{{'0','OFF',[]}},'TermMode',{{1,'OFF',[]}},'TLCFileName',{{'rtigensersetup','OFF',[]}})  RTISFcnParameters=struct('BoardNo','double','ChannelNo','double','ChannelNumOf','double','BaudRate','double','DataBitsNumOf','double','StopBitsNumOf','double','ParityMode','double','TransceiverMode','double','ReceiveIntLevelUart','double','AutoflowMode','double','FifoSize','double','ReceiveIntLevelFifo','double','FifoBlockSize','double','TermMode','double','QuartzFrequency','double','TLCFileName','char')  RTIBlockParaDefault=struct('ParityMode',1,'TransceiverMode',[1;1],'QuartzFrequency',160000000,'BoardNo',1,'ChannelNo',1,'ChannelNumOf',2,'BaudRate',115200,'DataBitsNumOf',4,'StopBitsNumOf',1,'ReceiveIntLevelUart',4,'AutoflowMode',0,'FifoSize',64,'ReceiveIntLevelFifo',0,'FifoOverrunMode',1,'FifoBlockSize',0,'TermMode',1,'TLCFileName','rtigensersetup')
  Data Store Memory : DataStoreMemory  DataStoreName=ExperimentCounterValue  WriteAfterWriteMsg=warning  ShowAdditionalParam=off
  Data Store Memory1 : DataStoreMemory  DataStoreName=last_curent  WriteAfterWriteMsg=warning  ShowAdditionalParam=off
  Data Store Memory10 : DataStoreMemory  DataStoreName=NumCountsPerSend  WriteAfterWriteMsg=warning  ShowAdditionalParam=off
  Data Store Memory11 : DataStoreMemory  DataStoreName=OutputReceived1  WriteAfterWriteMsg=warning  ShowAdditionalParam=off  OutDataTypeStr=double
  Data Store Memory12 : DataStoreMemory  DataStoreName=ObsSent  WriteAfterWriteMsg=warning  ShowAdditionalParam=off
  Data Store Memory13 : DataStoreMemory  DataStoreName=Counter  WriteAfterWriteMsg=warning  ShowAdditionalParam=off
  Data Store Memory14 : DataStoreMemory  DataStoreName=OutputReceived2  WriteAfterWriteMsg=warning  ShowAdditionalParam=off  OutDataTypeStr=double
  Data Store Memory15 : DataStoreMemory  DataStoreName=OutputReceived  WriteAfterWriteMsg=warning  ShowAdditionalParam=off  OutDataTypeStr=double
  Data Store Memory16 : DataStoreMemory  DataStoreName=last_state_lyap  WriteAfterWriteMsg=warning  InitialValue=[0,0,0,0,0,0,0,0,0,0]  ShowAdditionalParam=off  OutDataTypeStr=single  Dimensions=[10]
  Data Store Memory2 : DataStoreMemory  DataStoreName=last_disturbance  WriteAfterWriteMsg=warning  ShowAdditionalParam=off
  Data Store Memory3 : DataStoreMemory  DataStoreName=CRC_value  WriteAfterWriteMsg=warning  ShowAdditionalParam=off  OutDataTypeStr=uint8
  Data Store Memory4 : DataStoreMemory  DataStoreName=FlagStart  WriteAfterWriteMsg=warning  ShowAdditionalParam=off
  Data Store Memory5 : DataStoreMemory  DataStoreName=data_length  WriteAfterWriteMsg=warning  ShowAdditionalParam=off  OutDataTypeStr=uint8
  Data Store Memory6 : DataStoreMemory  DataStoreName=data_cmd_received  WriteAfterWriteMsg=warning  ShowAdditionalParam=off  OutDataTypeStr=uint8
  Data Store Memory7 : DataStoreMemory  DataStoreName=FlagAbort  WriteAfterWriteMsg=warning  ShowAdditionalParam=off  OutDataTypeStr=uint8
  Data Store Memory8 : DataStoreMemory  DataStoreName=FlagStartTrain  WriteAfterWriteMsg=warning  ShowAdditionalParam=off
  Data Store Memory9 : DataStoreMemory  DataStoreName=FlagReceivedAck  WriteAfterWriteMsg=warning  ShowAdditionalParam=off  OutDataTypeStr=uint8
  Data Store Read : DataStoreRead  DataStoreName=last_z_value  IndexOptions=Index vector (dialog)  Indices=1  OutputSizes=1
  Data Store Read1 : DataStoreRead  DataStoreName=last_z_value  IndexOptions=Index vector (dialog)  Indices=1  OutputSizes=1
  Data Store Read{2..4,9..10,13,16..17,20..23,27,34,37,39,41,43,51} (19 alike) : DataStoreRead  DataStoreName=StartSignalValue  IndexOptions=Index vector (dialog)  Indices=1  OutputSizes=1
  Data Store Read11 : DataStoreRead  DataStoreName=ExperimentCounterValue  IndexOptions=Index vector (dialog)  Indices=1  OutputSizes=1
  Data Store Read12 : DataStoreRead  DataStoreName=last_curent  IndexOptions=Index vector (dialog)  Indices=1  OutputSizes=1
  Data Store Read14 : DataStoreRead  DataStoreName=ExperimentCounterValue  IndexOptions=Index vector (dialog)  Indices=1  OutputSizes=1
  Data Store Read{6,15,18,24,30} (5 alike) : DataStoreRead  DataStoreName=RecordSignalValue  IndexOptions=Index vector (dialog)  Indices=1  OutputSizes=1
  Data Store Read{19,32,38,40,42,44} (6 alike) : DataStoreRead  DataStoreName=FlagStart  IndexOptions=Index vector (dialog)  Indices=1  OutputSizes=1
  Data Store Read25 : DataStoreRead  DataStoreName=last_curent  IndexOptions=Index vector (dialog)  Indices=1  OutputSizes=1
  Data Store Read26 : DataStoreRead  DataStoreName=last_disturbance  IndexOptions=Index vector (dialog)  Indices=1  OutputSizes=1
  Data Store Read28 : DataStoreRead  DataStoreName=last_z_value  IndexOptions=Index vector (dialog)  Indices=1  OutputSizes=1
  Data Store Read29 : DataStoreRead  DataStoreName=last_disturbance  IndexOptions=Index vector (dialog)  Indices=1  OutputSizes=1
  Data Store Read31 : DataStoreRead  DataStoreName=Counter  IndexOptions=Index vector (dialog)  Indices=1  OutputSizes=1
  Data Store Read33 : DataStoreRead  DataStoreName=NumCountsPerSend  IndexOptions=Index vector (dialog)  Indices=1  OutputSizes=1
  Data Store Read35 : DataStoreRead  DataStoreName=OutputReceived1  IndexOptions=Index vector (dialog)  Indices=1  OutputSizes=1
  Data Store Read36 : DataStoreRead  DataStoreName=OutputReceived2  IndexOptions=Index vector (dialog)  Indices=1  OutputSizes=1
  Data Store Read45 : DataStoreRead  DataStoreName=AmplitureRefSignal  IndexOptions=Index vector (dialog)  Indices=1  OutputSizes=1
  Data Store Read46 : DataStoreRead  DataStoreName=FreqRefSignal  IndexOptions=Index vector (dialog)  Indices=1  OutputSizes=1
  Data Store Read47 : DataStoreRead  DataStoreName=PosRandom  IndexOptions=Index vector (dialog)  Indices=1  OutputSizes=1
  Data Store Read48 : DataStoreRead  DataStoreName=PosRandom  IndexOptions=Index vector (dialog)  Indices=1  OutputSizes=1
  Data Store Read5 : DataStoreRead  DataStoreName=last_curent  IndexOptions=Index vector (dialog)  Indices=1  OutputSizes=1
  Data Store Read7 : DataStoreRead  DataStoreName=ExperimentCounterValue  IndexOptions=Index vector (dialog)  Indices=1  OutputSizes=1
  Data Store Read8 : DataStoreRead  DataStoreName=StartTimeSignal  IndexOptions=Index vector (dialog)  Indices=1  OutputSizes=1
  Data Store Write : DataStoreWrite  DataStoreName=last_z_value  IndexOptions=Index vector (dialog)  Indices=1  OutputSizes=1
  Data Store Write1 : DataStoreWrite  DataStoreName=StartSignalValue  IndexOptions=Index vector (dialog)  Indices=1  OutputSizes=1
  Data Store Write10 : DataStoreWrite  DataStoreName=RecordSignalValue  IndexOptions=Index vector (dialog)  Indices=1  OutputSizes=1
  Data Store Write11 : DataStoreWrite  DataStoreName=last_disturbance  IndexOptions=Index vector (dialog)  Indices=1  OutputSizes=1
  Data Store Write12 : DataStoreWrite  DataStoreName=last_z_value  IndexOptions=Index vector (dialog)  Indices=1  OutputSizes=1
  Data Store Write13 : DataStoreWrite  DataStoreName=last_disturbance  IndexOptions=Index vector (dialog)  Indices=1  OutputSizes=1
  Data Store Write14 : DataStoreWrite  DataStoreName=NumCountsPerSend  IndexOptions=Index vector (dialog)  Indices=1  OutputSizes=1
  Data Store Write15 : DataStoreWrite  DataStoreName=Counter  IndexOptions=Index vector (dialog)  Indices=1  OutputSizes=1
  Data Store Write16 : DataStoreWrite  DataStoreName=AmplitureRefSignal  IndexOptions=Index vector (dialog)  Indices=1  OutputSizes=1
  Data Store Write17 : DataStoreWrite  DataStoreName=FreqRefSignal  IndexOptions=Index vector (dialog)  Indices=1  OutputSizes=1
  Data Store Write18 : DataStoreWrite  DataStoreName=PosRandom  IndexOptions=Index vector (dialog)  Indices=1  OutputSizes=1
  Data Store Write19 : DataStoreWrite  DataStoreName=AmplitureRefSignal  IndexOptions=Index vector (dialog)  Indices=1  OutputSizes=1
  Data Store Write2 : DataStoreWrite  DataStoreName=RecordSignalValue  IndexOptions=Index vector (dialog)  Indices=1  OutputSizes=1
  Data Store Write3 : DataStoreWrite  DataStoreName=ExperimentCounterValue  IndexOptions=Index vector (dialog)  Indices=1  OutputSizes=1
  Data Store Write4 : DataStoreWrite  DataStoreName=ExperimentCounterValue  IndexOptions=Index vector (dialog)  Indices=1  OutputSizes=1
  Data Store Write5 : DataStoreWrite  DataStoreName=StartSignalValue  IndexOptions=Index vector (dialog)  Indices=1  OutputSizes=1
  Data Store Write6 : DataStoreWrite  DataStoreName=last_curent  IndexOptions=Index vector (dialog)  Indices=1  OutputSizes=1
  Data Store Write7 : DataStoreWrite  DataStoreName=ExperimentCounterValue  IndexOptions=Index vector (dialog)  Indices=1  OutputSizes=1
  Data Store Write8 : DataStoreWrite  DataStoreName=StartSignalValue  IndexOptions=Index vector (dialog)  Indices=1  OutputSizes=1
  Data Store Write9 : DataStoreWrite  DataStoreName=RecordSignalValue  IndexOptions=Index vector (dialog)  Indices=1  OutputSizes=1
  DataReceiveStep : DataStoreMemory  DataStoreName=DataReceiveStep  WriteAfterWriteMsg=warning  ShowAdditionalParam=off  OutDataTypeStr=uint8
  Discrete Derivative1 : simulink/Discrete/Discrete Derivative  gainval=1.0  ICPrevScaledInput=0.0  OutMin=[]  OutMax=[]  OutDataType=fixdt(1, 16)  OutScaling=2^-10  DoSatur=off
  Discrete Derivative3 : simulink/Discrete/Discrete Derivative  gainval=1.0  ICPrevScaledInput=0.0  OutMin=[]  OutMax=[]  OutDataType=fixdt(1, 16)  OutScaling=2^-10  DoSatur=off
  Discrete-Time Integrator : DiscreteIntegrator  ExternalReset=falling  SampleTime=-1  ICPrevOutput=DiscIntNeverNeededParam  ICPrevScaledInput=DiscIntNeverNeededParam
  Discrete-Time Integrator1 : DiscreteIntegrator  ExternalReset=falling  SampleTime=-1  ICPrevOutput=DiscIntNeverNeededParam  ICPrevScaledInput=DiscIntNeverNeededParam
  Discrete-Time Integrator2 : DiscreteIntegrator  ExternalReset=either  SampleTime=-1  ICPrevOutput=DiscIntNeverNeededParam  ICPrevScaledInput=DiscIntNeverNeededParam
  Discrete-Time Integrator3 : DiscreteIntegrator  ExternalReset=falling  SampleTime=-1  ICPrevOutput=DiscIntNeverNeededParam  ICPrevScaledInput=DiscIntNeverNeededParam
  Discrete-Time Integrator4 : DiscreteIntegrator  ExternalReset=either  SampleTime=-1  ICPrevOutput=DiscIntNeverNeededParam  ICPrevScaledInput=DiscIntNeverNeededParam
  DiscreteContinousMode : Constant
  DisturbanceEstimationPhase1 : MATLAB Function  TreatAsAtomicUnit=on
  DisturbanceEstimationPhase2 : MATLAB Function  TreatAsAtomicUnit=on
  DisturbanceFormulationModelValue : Constant  Value=2
  DisturbanceMultiplier : Constant  Value=0
  Divide{,1..3} (4 alike) : Product  Inputs=*/
  EMC_ENCODER_BL1 : rtiemclib/EMC_ENCODER_BL1  DSProperties=struct('RTI',struct('Version',uint32(2),'BlockType',struct('isSLSource',uint8(1),'isSLSink',uint8(0),'isHWSource',uint8(1),'isHWSink',uint8(0),'isSetup',uint8(0),'isInline',uint8(1),'isNonInline',uint8(0),'isInterrupt',uint8(0),'isChannelwise',uint8(1)),'IOBoardType','DSEMC','UnitType','ENCODER','Identifier','ENCODER','DialogType','ML','BlockSet','RTIEMC','SlaveProcessor','NONE'))  RTIBlockInterface=struct('OutputPortsWidth',int32([1 1 1]),'OutputPortsActive',int32([1 1 0]),'OutputPortsName',{{'Position','Speed',['Index Detected']}},'OutputPortsDataType',{{'SS_DOUBLE','SS_DOUBLE','SS_BOOLEAN'}},'InitLevel',3,'IconTransparency','on','BlockDisplay',{{['EMC Encoder\nUnit: 5\nDIO class: 1\nPort: 3\nChannel: 10'],'center'}},'DialogFcn','rtiemcencodergui','BlockName',struct('Token',{{'EMC_ENCODER_BL1'}}))  RTIBlockParameters=struct('UnitNo',{{5,'OFF',[1 6]}},'DioClassNo',{{1,'OFF',[1 2]}},'PortNo',{{3,'OFF',[1 3]}},'ChannelNo',{{10,'OFF',[1 15]}},'HwSignalPin',{{['DIO1 ch1'],'OFF',[]}},'HwRefPin',{{'GND','OFF',[]}},'EnablePosMeasurement',{{0,'OFF',[0 1]}},'IndexSetMode',{{1,'OFF',[1 3]}},'EnableMinSpeed',{{0,'OFF',[0 1]}},'NumOfLines',{{'1024000','OFF',[1 2097152]}},'InitAngleValue',{{'0','OFF',[0 359.99999]}},'IndexAngleValue',{{'0','OFF',[0 359.99999]}},'MinSpeedAngleValue',{{'45','OFF',[0.01 1464.84]}},'MinPosValue',{{'0','OFF',[-2097152 2097150.75]}},'MaxPosValue',{{'1023.75','OFF',[-2097151 2097151.75]}},'InitPosValue',{{'0','OFF',[-2097152 2097151.75]}},'IndexPosValue',{{'0','OFF',[-2097152 2097151.75]}},'MinSpeedPosValue',{{'100','OFF',[1 1000000]}},'IndexGateMode',{{0,'OFF',[0 1]}},'EnableNoiseFilter',{{0,'OFF',[0 1]}},'FilterInterval',{{'0','OFF',[0 0.01]}},'IndexDetectedOutPortMode',{{0,'OFF',[0 1]}},'BuildCheckAngleMeasurement',{{1,'OFF',[0 1]}},'BuildCheckAngleIndexMode',{{0,'OFF',[0 1]}},'BuildCheckPosIndexMode',{{0,'OFF',[0 1]}},'BuildCheckAngleMinSpeed',{{0,'OFF',[0 1]}},'BuildCheckPosMinSpeed',{{0,'OFF',[0 1]}},'TLCFileName',{{'rtiemcencoder','OFF',[]}})  RTISFcnParameters=struct('UnitNo','int32','DioClassNo','int32','PortNo','int32','ChannelNo','int32','EnablePosMeasurement','int32','IndexSetMode','int32','IndexDetectedOutPortMode','int32','EnableMinSpeed','int32','NumOfLines','uint32','InitAngleValue','double','IndexAngleValue','double','MinSpeedAngleValue','double','MinPosValue','double','MaxPosValue','double','InitPosValue','double','IndexPosValue','double','MinSpeedPosValue','double','IndexGateMode','int32','EnableNoiseFilter','int32','FilterInterval','double','TLCFileName','char')  RTIBlockParaDefault=struct('UnitNo',1,'DioClassNo',1,'PortNo',1,'ChannelNo',1,'HwSignalPin',['DIO1 ch1'],'HwRefPin','GND','EnablePosMeasurement',0,'IndexSetMode',1,'EnableMinSpeed',0,'NumOfLines',1024,'InitAngleValue',60,'IndexAngleValue',0,'MinSpeedAngleValue',45,'MinPosValue',0,'MaxPosValue',1023.75,'InitPosValue',0,'IndexPosValue',0,'MinSpeedPosValue',100,'IndexGateMode',0,'EnableNoiseFilter',0,'FilterInterval',0,'IndexDetectedOutPortMode',0,'BuildCheckAngleMeasurement',1,'BuildCheckAngleIndexMode',0,'BuildCheckPosIndexMode',0,'BuildCheckAngleMinSpeed',0,'BuildCheckPosMinSpeed',0,'TLCFileName','rtiemcencoder')
      settings: SourceProductName=dSPACE RTI Electric Motor Control Blockset
  EMC_ENCODER_BL2 : rtiemclib/EMC_ENCODER_BL1  DSProperties=struct('RTI',struct('Version',uint32(2),'BlockType',struct('isSLSource',uint8(1),'isSLSink',uint8(0),'isHWSource',uint8(1),'isHWSink',uint8(0),'isSetup',uint8(0),'isInline',uint8(1),'isNonInline',uint8(0),'isInterrupt',uint8(0),'isChannelwise',uint8(1)),'IOBoardType','DSEMC','UnitType','ENCODER','Identifier','ENCODER','DialogType','ML','BlockSet','RTIEMC','SlaveProcessor','NONE'))  RTIBlockInterface=struct('OutputPortsWidth',int32([1 1 1]),'OutputPortsActive',int32([1 1 0]),'OutputPortsName',{{'Position','Speed',['Index Detected']}},'OutputPortsDataType',{{'SS_DOUBLE','SS_DOUBLE','SS_BOOLEAN'}},'InitLevel',3,'IconTransparency','on','BlockDisplay',{{['EMC Encoder\nUnit: 1\nDIO class: 1\nPort: 3\nChannel: 15'],'center'}},'DialogFcn','rtiemcencodergui','BlockName',struct('Token',{{'EMC_ENCODER_BL1'}}))  RTIBlockParameters=struct('UnitNo',{{1,'OFF',[1 6]}},'DioClassNo',{{1,'OFF',[1 2]}},'PortNo',{{3,'OFF',[1 3]}},'ChannelNo',{{15,'OFF',[1 15]}},'HwSignalPin',{{['DIO1 ch1'],'OFF',[]}},'HwRefPin',{{'GND','OFF',[]}},'EnablePosMeasurement',{{1,'OFF',[0 1]}},'IndexSetMode',{{1,'OFF',[1 3]}},'EnableMinSpeed',{{0,'OFF',[0 1]}},'NumOfLines',{{'10240','OFF',[1 2097152]}},'InitAngleValue',{{'0','OFF',[0 359.99999]}},'IndexAngleValue',{{'0','OFF',[0 359.99999]}},'MinSpeedAngleValue',{{'45','OFF',[0.01 10000]}},'MinPosValue',{{'-1000000','OFF',[-2097152 2097150.75]}},'MaxPosValue',{{'1000000.75','OFF',[-2097151 2097151.75]}},'InitPosValue',{{'0','OFF',[-2097152 2097151.75]}},'IndexPosValue',{{'0','OFF',[-2097152 2097151.75]}},'MinSpeedPosValue',{{'100','OFF',[1 1000000]}},'IndexGateMode',{{0,'OFF',[0 1]}},'EnableNoiseFilter',{{0,'OFF',[0 1]}},'FilterInterval',{{'0','OFF',[0 0.01]}},'IndexDetectedOutPortMode',{{0,'OFF',[0 1]}},'BuildCheckAngleMeasurement',{{0,'OFF',[0 1]}},'BuildCheckAngleIndexMode',{{0,'OFF',[0 1]}},'BuildCheckPosIndexMode',{{0,'OFF',[0 1]}},'BuildCheckAngleMinSpeed',{{0,'OFF',[0 1]}},'BuildCheckPosMinSpeed',{{0,'OFF',[0 1]}},'TLCFileName',{{'rtiemcencoder','OFF',[]}})  RTISFcnParameters=struct('UnitNo','int32','DioClassNo','int32','PortNo','int32','ChannelNo','int32','EnablePosMeasurement','int32','IndexSetMode','int32','IndexDetectedOutPortMode','int32','EnableMinSpeed','int32','NumOfLines','uint32','InitAngleValue','double','IndexAngleValue','double','MinSpeedAngleValue','double','MinPosValue','double','MaxPosValue','double','InitPosValue','double','IndexPosValue','double','MinSpeedPosValue','double','IndexGateMode','int32','EnableNoiseFilter','int32','FilterInterval','double','TLCFileName','char')  RTIBlockParaDefault=struct('UnitNo',1,'DioClassNo',1,'PortNo',1,'ChannelNo',1,'HwSignalPin',['DIO1 ch1'],'HwRefPin','GND','EnablePosMeasurement',0,'IndexSetMode',1,'EnableMinSpeed',0,'NumOfLines',1024,'InitAngleValue',60,'IndexAngleValue',0,'MinSpeedAngleValue',45,'MinPosValue',0,'MaxPosValue',1023.75,'InitPosValue',0,'IndexPosValue',0,'MinSpeedPosValue',100,'IndexGateMode',0,'EnableNoiseFilter',0,'FilterInterval',0,'IndexDetectedOutPortMode',0,'BuildCheckAngleMeasurement',1,'BuildCheckAngleIndexMode',0,'BuildCheckPosIndexMode',0,'BuildCheckAngleMinSpeed',0,'BuildCheckPosMinSpeed',0,'TLCFileName','rtiemcencoder')
      settings: SourceProductName=dSPACE RTI Electric Motor Control Blockset
  Edge Detector : spsEdgeDetectorLib/Edge Detector  model=Either  ic=0  Ts=0
      settings: LibrarySourceBlock=sps_lib/Control/Edge Detector
  Edge Detector1 : spsEdgeDetectorLib/Edge Detector  model=Rising  ic=0  Ts=0
      settings: LibrarySourceBlock=sps_lib/Control/Edge Detector
  Edge Detector2 : spsEdgeDetectorLib/Edge Detector  model=Falling  ic=0  Ts=0
      settings: LibrarySourceBlock=sps_lib/Control/Edge Detector
  Edge Detector3 : spsEdgeDetectorLib/Edge Detector  model=Falling  ic=0  Ts=0
      settings: LibrarySourceBlock=sps_lib/Control/Edge Detector
  Edge Detector4 : spsEdgeDetectorLib/Edge Detector  model=Rising  ic=0  Ts=0
      settings: LibrarySourceBlock=sps_lib/Control/Edge Detector
  Enc2CorrectionFactor : Constant  Value=1.25
  Enc2StartPosition : Constant  Value=1*0.054
  ExperimentTime : Constant  Value=50
  FLcontroller : MATLAB Function  TreatAsAtomicUnit=on
  FLcontroller1 : MATLAB Function  TreatAsAtomicUnit=on
  FilterConstant : Constant  Value=0.00004
  FlagWriteStartTimeSignalBlock : Constant  Value=0
  ForceHydOffset : Constant  Value=-30
  ForceLoadOffset : Constant  Value=-30
  FreqRefSignalMemory : DataStoreMemory  DataStoreName=FreqRefSignal  WriteAfterWriteMsg=warning  ShowAdditionalParam=off
  FreqRefSignalMemory1 : DataStoreMemory  DataStoreName=PosRandom  WriteAfterWriteMsg=warning  ShowAdditionalParam=off
  FreqRefSignalRead : DataStoreRead  DataStoreName=FreqRefSignal  IndexOptions=Index vector (dialog)  Indices=1  OutputSizes=1
  FreqRefSignalRead1 : DataStoreRead  DataStoreName=FreqRefSignal  IndexOptions=Index vector (dialog)  Indices=1  OutputSizes=1
  FreqRefSignalValue : Constant
  FunctionCalculateHydModel : MATLAB Function  TreatAsAtomicUnit=on
  Gain : Gain  Gain=((1/6250)*2.032)/1000
  Gain1 : Gain
  Gain2 : Gain  Gain=str2num(get_param('Teste_PID/Enc2CorrectionFactor','Value'))*10
  Gain3 : Gain  Gain=-1
  GainRampDist1 : Constant  Value=16
  GainRampDist2 : Constant  Value=64
  GainRampDist3 : Constant  Value=0
  GradConst : Constant  Value=0.0001
  IntegralMemory : DataStoreMemory  DataStoreName=IntegralMemoryValue  WriteAfterWriteMsg=warning  ShowAdditionalParam=off
  Interrupt-Driven Reception : Subsystem  TreatAsAtomicUnit=on
  Kd_value : Constant  Value=0
  Kd_value1 : Constant  Value=0
  Ki_value : Constant  Value=5
  Ki_value1 : Constant  Value=10
  Kp_value : Constant  Value=15
  Kp_value1 : Constant  Value=15
  LengthCylinder : Constant  Value=0.08
  Low-Pass Filter (Discrete or Continuous){,2..8} (8 alike) : eeGeneralControl/Low-Pass Filter (Discrete or Continuous)  K=1  T=str2num(get_param('Teste_PID/FilterConstant','Value'))  B=inf  A=-inf  init_option=Inherited from block input  x0=0  Ts=-1
  MATLAB Function : MATLAB Function  TreatAsAtomicUnit=on
  MATLAB Function1 : MATLAB Function  TreatAsAtomicUnit=on
  MATLAB Function2 : MATLAB Function  TreatAsAtomicUnit=on
  MATLAB Function4 : MATLAB Function  TreatAsAtomicUnit=on
  MATLAB Sweep : MATLAB Function  TreatAsAtomicUnit=on
  MaxFreq : Constant  Value=2.5
  Mux : Mux  Inputs=8
  NumberExperiments : Constant
  PID_FL_Value : Constant  Value=0
  Pn : Constant  Value=7000000
  PolyDerivativeSubSystem1 : Subsystem
  PolyDerivativeSubSystem2 : Subsystem
  PolyDerivativeSubSystem3 : Subsystem
  PolyDerivativeSubSystem4 : Subsystem
  PolyDerivativeSubSystem5 : Subsystem
  PolyDerivativeSubSystem6 : Subsystem
  Product : Product  Inputs=3
  Product{1..8,10..18,20} (18 alike) : Product
  Qn : Constant  Value=10/60000
  RLAction : Scope
  RL_FL : MATLAB Function  TreatAsAtomicUnit=on
  RLgain : Constant
  RTI Data : Subsystem  Tag=struct('RTIDataServer',struct('RTIDataServerVs','2','RTIModelDescription','struct(''main'',''Teste_PID'',''sub'','''',''isMp'',0)'))  LoadFcn="if exist('rtidc'), try,  rtidc('DataHostBlockClbLoad', gcbh); catch, disp(['Warning: ''LoadFcn'' for RTI Data block failed: ' lasterr]); end, end,"  mask(RTI_DATA_HOST){}
      mask help:
      | RTI Data Block.
      | This block is used by RTI to store internal model-dependent data.
      | Please keep this block on the root level of the model. Deleting this block will result in data loss.
      |
      | NEVER DELETE OR COPY THIS BLOCK!
      settings: CopyFcn="if exist('rtidc'), try,  rtidc('DataHostBlockClbCopy', gcbh); catch, disp(['Warning: ''CopyFcn'' for RTI Data block failed: ' lasterr]); end, end,"  DeleteFcn="if exist('rtidc'), try,  rtidc('DataHostBlockClbDelete', gcbh); catch, disp(['Warning: ''DeleteFcn'' for RTI Data block failed: ' lasterr]); end, end,"  ModelCloseFcn="if exist('rtidc'), try,  rtidc('DataHostBlockClbModelClose', gcbh); catch, disp(['Warning: ''ModelCloseFcn'' for RTI Data block failed: ' lasterr]); end, end,"  PreSaveFcn="if exist('rtidc'), try,  rtidc('DataHostBlockClbPreSave', gcbh); catch, disp(['Warning: ''PreSaveFcn'' for RTI Data block failed: ' lasterr]); end, end,"  PostSaveFcn="if exist('rtidc'), try,  rtidc('DataHostBlockClbPostSave', gcbh); catch, disp(['Warning: ''PostSaveFcn'' for RTI Data block failed: ' lasterr]); end, end,"  NameChangeFcn="if exist('rtidc'), try,  rtidc('DataHostBlockClbNameChange', gcbh); catch, disp(['Warning: ''NameChangeFcn'' for RTI Data block failed: ' lasterr]); end, end,"
      mask Help:
      | RTI Data Block.
      | This block is used by RTI to store internal model-dependent data.
      | Please keep this block on the root level of the model. Deleting this block will result in data loss.
      | 
      | NEVER DELETE OR COPY THIS BLOCK!
      mask Display:
      | text(0.5, 0.5, 'RTI Data', 'HorizontalAlignment', 'center');
      | plot([1 0]);
  Random : Constant  Value=0
  RecordSignalValueMemory : DataStoreMemory  DataStoreName=RecordSignalValue  WriteAfterWriteMsg=warning  ShowAdditionalParam=off
  RefFunctionSin : MATLAB Function  TreatAsAtomicUnit=on
  RefRand : MATLAB Function  TreatAsAtomicUnit=on
  RefStepFunction : MATLAB Function  TreatAsAtomicUnit=on
  Saturation : Saturate  UpperLimit=str2num(get_param('Teste_PID/Un','Value'))/str2num(get_param('Teste_PID/SaturationDivider','Value'))  LowerLimit=-str2num(get_param('Teste_PID/Un','Value'))/str2num(get_param('Teste_PID/SaturationDivider','Value'))
  Saturation1 : Saturate  UpperLimit=0.0008  LowerLimit=-0.0008
  Saturation3 : Saturate  UpperLimit=str2num(get_param('Teste_PID/Un','Value'))/str2num(get_param('Teste_PID/SaturationDivider','Value'))  LowerLimit=-str2num(get_param('Teste_PID/Un','Value'))/str2num(get_param('Teste_PID/SaturationDivider','Value'))
  Saturation4 : Saturate  UpperLimit=str2num(get_param('Teste_PID/Un','Value'))/str2num(get_param('Teste_PID/SaturationDivider','Value'))  LowerLimit=-str2num(get_param('Teste_PID/Un','Value'))/str2num(get_param('Teste_PID/SaturationDivider','Value'))
  Saturation6 : Saturate  UpperLimit=1  LowerLimit=-1
  SaturationDivider : Constant
  Scope{,1..2,5} (4 alike) : Scope
  ScopeControl : Scope
  ScopeCounter : Scope
  ScopeDRefSignal : Scope
  ScopeEdge : Scope
  ScopeFlagStart : Scope
  ScopeForceError : Scope
  ScopeForceError1 : Scope
  ScopeKiRl : Scope
  ScopeKpRl : Scope
  ScopeOutput : Scope
  ScopePID : Scope
  ScopePID1 : Scope
  ScopeRecordingSignal : Scope
  ScopeRefSignal : Scope
  Scope_DForce_Hyd : Scope
  Scope_DForce_Load : Scope
  Scope_DForce_Load_Old : Scope
  Scope_Disturbance : Scope
  Scope_Force_Hyd : Scope
  Scope_Force_Hyd_Filter : Scope
  Scope_Force_Load : Scope
  Scope_Force_Load_Filter : Scope
  Scope_Pa : Scope
  Scope_Pa_Filter : Scope
  Scope_Pb : Scope
  Scope_Pb_Filter : Scope
  Scope_Pos1 : Scope
  Scope_Pos1_Filter : Scope
  Scope_Pos2 : Scope
  Scope_Pos2_Filter : Scope
  Scope_Psource : Scope
  Scope_Psource_Filter : Scope
  Scope_Ptank : Scope
  Scope_Ptank_Filter : Scope
  Scope_SpringForce : Scope
  Scope_d_force_model : Scope
  Scope_f_hyd_model : Scope
  Scope_g_hyd_model : Scope
  SetStartTime : MATLAB Function  TreatAsAtomicUnit=on
  SimTimeMemory : DataStoreMemory  DataStoreName=SimTimeSignal  WriteAfterWriteMsg=warning  ShowAdditionalParam=off
  SimTimeSignalRead{,1..5} (6 alike) : DataStoreRead  DataStoreName=SimTimeSignal  IndexOptions=Index vector (dialog)  Indices=1  OutputSizes=1
  SimTimeWrite : DataStoreWrite  DataStoreName=SimTimeSignal  IndexOptions=Index vector (dialog)  Indices=1  OutputSizes=1
  SineStepRefSignalValue : Constant  Value=0
  SmoothFactor : Constant  Value=0
  StartSignaMemory : DataStoreMemory  DataStoreName=StartSignalValue  WriteAfterWriteMsg=warning  ShowAdditionalParam=off
  StartStopRecordingController : MATLAB Function  TreatAsAtomicUnit=on
  StartTimeSignalMemory : DataStoreMemory  DataStoreName=StartTimeSignal  WriteAfterWriteMsg=warning  ShowAdditionalParam=off
  StartTimeSignalRead{,1..4} (5 alike) : DataStoreRead  DataStoreName=StartTimeSignal  IndexOptions=Index vector (dialog)  Indices=1  OutputSizes=1
  StartTimeSignalWrite : DataStoreWrite  DataStoreName=StartTimeSignal  IndexOptions=Index vector (dialog)  Indices=1  OutputSizes=1
  Sum : Sum  Inputs=|-+
  Sum1 : Sum  Inputs=|+-
  Sum{2,5..7} (4 alike) : Sum  Inputs=|++
  Sum3 : Sum  Inputs=|+++
  Sum4 : Sum  Inputs=|-+
  Sum8 : Sum  Inputs=|+++
  Switch : Switch  Criteria=u2 > Threshold  SaturateOnIntegerOverflow=off  InputSameDT=off
  Switch1 : Switch  Criteria=u2 > Threshold  SaturateOnIntegerOverflow=off  InputSameDT=off
  TimerValue : Constant  Value=0.00001
  Un : Constant  Value=0.05
  Vpl : Constant  Value=0.00121
  Vpl_old : Constant  Value=0.004*0.004*3.1415*0.25*0.95
  controller_select : Constant  Value=0
  lambda_value : Constant  Value=0
  last_z_valueMemory : DataStoreMemory  DataStoreName=last_z_value  WriteAfterWriteMsg=warning  ShowAdditionalParam=off
  start_freq : Constant  Value=0.5
  tag scope: Alpha=global, Ap=global, Be=global, C1=global, C2=global, ControlAction=global, ControllerSelect=global, DDPosEnc2=global, DForce_Hyd=global, DForce_Load=global, DPosEnc2=global, DReference=global, DiscreteContinousMode=global, Force_Hyd=global, Force_Load=global, GradConst=global, Kd=global, Kd_Pos=global, Ki=global, KiRl=global, Ki_Pos=global, Kp=global, KpRl=global, Kp_Pos=global, LastAction=global, LastAction_RL=global, Lcy=global, Pa=global, Pb=global, Pn=global, PolyFitPoints=global, PosEnc2=global, Qn=global, Reference=global, SmoothFactor=global, Un=global, Vpl=global, leak=global
  wires:
  SetStartTime/1(start_time) -> StartTimeSignalWrite/1
  StartTimeSignalRead1/1 -> SetStartTime/3(start)
  SimTimeSignalRead/1 -> RefFunctionSin/1(Time)
  SimTimeSignalRead1/1 -> SetStartTime/2(time)
  FreqRefSignalRead/1 -> RefFunctionSin/3(Freq)
  StartTimeSignalRead/1 -> RefFunctionSin/4(StartTime)
  Clock/1 -> SimTimeWrite/1
  Edge Detector/1 -> ScopeEdge/1, SetStartTime/1(flag)
  AmplitureRefSignalRead/1 -> RefFunctionSin/2(Amp)
  lambda_value/1 -> [lambda]
  Kp_value/1 -> [Kp]
  Ki_value/1 -> [Ki]
  Kd_value/1 -> [Kd]
  Pn/1 -> [Pn]
  Un/1 -> [Un]
  Qn/1 -> [Qn]
  Bulk/1 -> [Be]
  CylinderArea/1 -> [Ap]
  CylinderAreaRatio/1 -> [Alpha]
  LengthCylinder/1 -> [Lcy]
  [Force_Load] -> Sum/1
  [Reference] -> Sum/2
  Sum/1 -> ScopeForceError/1, Product3/1, PolyDerivativeSubSystem6/1(Signal), [ForceError]
  PolyDerivativeSubSystem6/1(dSignal) -> [DForceError]
  Discrete-Time Integrator2/1 -> [IntForceError]
  FunctionCalculateHydModel/1(f) -> [f_HydMode], Scope_f_hyd_model/1
  [Pn] -> FunctionCalculateHydModel/2(Pn)
  [Qn] -> FunctionCalculateHydModel/3(Qn)
  [Un] -> FunctionCalculateHydModel/4(Un)
  [Vpl] -> FunctionCalculateHydModel/5(Vpl)
  [PosEnc2] -> FunctionCalculateHydModel/6(xp)
  [Pa] -> FunctionCalculateHydModel/7(Pa)
  [Pb] -> FunctionCalculateHydModel/8(Pb)
  Constant6/1 -> FunctionCalculateHydModel/9(Ps)
  Constant/1 -> FunctionCalculateHydModel/10(Pt)
  [DPosEnc2] -> FunctionCalculateHydModel/11(xpd)
  [Lcy] -> FunctionCalculateHydModel/12(L_cyl)
  [Ap] -> FunctionCalculateHydModel/13(Aa)
  [Alpha] -> FunctionCalculateHydModel/14(alfa)
  C1/1 -> [C1]
  C2/1 -> [C2]
  [C1] -> FunctionCalculateHydModel/15(c1)
  [C2] -> FunctionCalculateHydModel/16(c2)
  [Be] -> FunctionCalculateHydModel/17(Be)
  RefFunctionSin/1(y) -> Switch/1, Switch/3
  Switch/1 -> Product/1
  SineStepRefSignalValue/1 -> [SineStepRefSignal]
  [SineStepRefSignal] -> Switch/2
  SimTimeSignalRead2/1 -> RefStepFunction/1(Time)
  AmplitureRefSignalRead1/1 -> RefStepFunction/2(Amp)
  StartTimeSignalRead2/1 -> RefStepFunction/3(StartTime)
  PID_FL_Value/1 -> [PID_FL_ValueSignal]
  Discrete Derivative3/1 -> [DReference], ScopeDRefSignal/1
  [f_HydMode] -> FLcontroller/2(f)
  [g_HydModel] -> FLcontroller/3(g)
  [DReference] -> FLcontroller/4(dFref)
  [PID_Value] -> FLcontroller/1(pid)
  DisturbanceEstimationPhase1/1(dz) -> Discrete-Time Integrator3/1
  [f_HydMode] -> DisturbanceEstimationPhase1/1(f)
  [g_HydModel] -> DisturbanceEstimationPhase1/2(g)
  Data Store Read12/1 -> DisturbanceEstimationPhase1/3(current)
  [lambda] -> DisturbanceEstimationPhase1/4(lambda)
  [Force_Load] -> DisturbanceEstimationPhase1/5(F)
  Data Store Read/1 -> DisturbanceEstimationPhase1/6(z)
  Discrete-Time Integrator3/1 -> Data Store Write/1, DisturbanceEstimationPhase2/4(z)
  [f_HydMode] -> DisturbanceEstimationPhase2/3(F)
  [lambda] -> DisturbanceEstimationPhase2/2(lambda)
  [g_HydModel] -> DisturbanceEstimationPhase2/1(g)
  DisturbanceEstimationPhase2/1(d) -> Product2/2
  [Disturbance] -> FLcontroller/5(d)
  DisturbanceFormulationModelValue/1 -> [DisturbanceFormulationSignal]
  GainRampDist1/1 -> [GainRampDist1Value]
  GainRampDist2/1 -> [GainRampDist2Value]
  [Force_Load] -> Divide/1
  [g_HydModel] -> Divide/2
  Divide/1 -> Sum1/1
  Data Store Read1/1 -> Sum1/2
  Discrete-Time Integrator1/1 -> Discrete-Time Integrator/1, [int_Fg_menos_z]
  [DisturbanceFormulationSignal] -> DisturbanceEstimationPhase1/7(dist_model)
  [GainRampDist1Value] -> DisturbanceEstimationPhase1/8(gain1)
  [GainRampDist2Value] -> DisturbanceEstimationPhase1/9(gain2)
  [Fg_menos_z] -> DisturbanceEstimationPhase1/10(Fmenos_z)
  [int_Fg_menos_z] -> DisturbanceEstimationPhase1/11(intFmenos_z)
  [DForce_Load] -> DisturbanceEstimationPhase1/12(dFF)
  DisturbanceMultiplier/1 -> [DisturbanceMultiplierValue]
  [DisturbanceMultiplierValue] -> Product2/1
  [DisturbanceFormulationSignal] -> DisturbanceEstimationPhase2/5(dist_model)
  [GainRampDist1Value] -> DisturbanceEstimationPhase2/6(gain1)
  [GainRampDist2Value] -> DisturbanceEstimationPhase2/7(gain2)
  [Fg_menos_z] -> DisturbanceEstimationPhase2/8(Fmenos_z)
  [int_Fg_menos_z] -> DisturbanceEstimationPhase2/9(intFmenos_z)
  NumberExperiments/1 -> [NumberExperimentsValue]
  ExperimentTime/1 -> [ExperimentTimeValue]
  [ExperimentTimeValue] -> RefStepFunction/4(EndTime)
  [ExperimentTimeValue] -> RefFunctionSin/5(EndTime)
  Data Store Read4/1 -> Product1/2
  Data Store Read3/1 -> Product/2
  [FlagWriteStartTimeSignalValue] -> Edge Detector1/1
  FlagWriteStartTimeSignalBlock/1 -> [FlagWriteStartTimeSignalValue]
  Data Store Read42/1 -> Edge Detector/1, ScopeRecordingSignal/1
  Data Store Read2/1 -> StartStopRecordingController/1(start_signal_value)
  Data Store Read6/1 -> StartStopRecordingController/2(recording_signal_value)
  Data Store Read7/1 -> StartStopRecordingController/3(counter_value)
  Data Store Read8/1 -> StartStopRecordingController/4(start_time)
  [ExperimentTimeValue] -> StartStopRecordingController/6(experiment_time_value)
  [NumberExperimentsValue] -> StartStopRecordingController/5(number_experiments)
  StartStopRecordingController/1(start_signal_value_update) -> Data Store Write1/1
  StartStopRecordingController/2(recording_signal_value_update) -> Data Store Write2/1
  StartStopRecordingController/3(counter_value_update) -> Data Store Write3/1
  SimTimeSignalRead3/1 -> StartStopRecordingController/7(time)
  Edge Detector1/1 -> MATLAB Function/1(edge)
  MATLAB Function/1(y) -> Scope/1, Data Store Write5/1
  Data Store Read10/1 -> MATLAB Function/2(last_value)
  Data Store Read11/1 -> MATLAB Function/3(last_value_counter)
  MATLAB Function/2(v) -> Data Store Write4/1
  Product1/1 -> Saturation/1
  Saturation/1 -> ScopeControl/1, Divide1/1
  [Un] -> Divide1/2
  Data Store Read5/1 -> FunctionCalculateHydModel/1(ixv)
  Data Store Read13/1 -> MATLAB Function1/2(last_value)
  Edge Detector2/1 -> MATLAB Function1/1(edge)
  MATLAB Function1/1(y) -> Data Store Write8/1, Scope2/1
  [FlagWriteStartTimeSignalValue] -> Edge Detector2/1
  MATLAB Function1/2(v) -> Data Store Write7/1
  Data Store Read14/1 -> MATLAB Function1/3(last_value_counter)
  Product5/1 -> Sum3/2
  [DForceError] -> Product7/2
  Product7/1 -> Sum3/3
  Product6/1 -> Sum3/1
  Sum3/1 -> Product4/1
  [ForceError] -> Product5/1
  Product3/1 -> Discrete-Time Integrator2/1
  Data Store Read17/1 -> Product3/2
  [Kp] -> Product5/2
  Product4/1 -> [PID_Value], ScopePID/1
  Data Store Read16/1 -> Product4/2
  [Ki] -> Product6/1
  [Kd] -> Product7/1
  Data Store Read19/1 -> Discrete-Time Integrator2/2
  [IntForceError] -> Product6/2
  Data Store Read15/1 -> Discrete-Time Integrator1/2, Discrete-Time Integrator/2
  Data Store Read20/1 -> FunctionCalculateHydModel/18(flag_start)
  Data Store Read21/1 -> DisturbanceEstimationPhase1/13(flag_start)
  Data Store Read22/1 -> DisturbanceEstimationPhase2/10(flag_start)
  Data Store Read23/1 -> FLcontroller/6(flag_start)
  Data Store Read18/1 -> MATLAB Function1/4(last_value_recording)
  MATLAB Function1/3(x) -> Data Store Write9/1
  Data Store Read24/1 -> MATLAB Function/4(last_value_recording)
  MATLAB Function/3(x) -> Data Store Write10/1
  Gain3/1 -> DAC_CLASS1_BL1/1
  FunctionCalculateHydModel/2(g) -> [g_HydModel], Scope_g_hyd_model/1
  FunctionCalculateHydModel/3(dF_model) -> Scope_d_force_model/1, [D_Force_Model]
  Data Store Read25/1 -> FunctionCalculateHydModel/20(current)
  Data Store Read26/1 -> FunctionCalculateHydModel/19(d)
  Data Store Read27/1 -> Product8/2
  Sum1/1 -> Product8/1
  Product8/1 -> Discrete-Time Integrator1/1, [Fg_menos_z]
  Data Store Read29/1 -> MATLAB Function/5(last_value_disturb)
  Data Store Read28/1 -> MATLAB Function/6(last_value_z)
  MATLAB Function/4(w) -> Data Store Write13/1
  MATLAB Function/5(e) -> Data Store Write12/1
  Discrete-Time Integrator/1 -> [int_int_Fg_menos_z]
  FLcontroller/1(y) -> Product1/1
  Data Store Read30/1 -> Discrete-Time Integrator3/2
  Product2/1 -> Scope_Disturbance/1, Saturation1/1
  Saturation1/1 -> Data Store Write11/1, [Disturbance]
  Vpl/1 -> [Vpl]
  GainRampDist3/1 -> [GainRampDist3Value]
  [int_int_Fg_menos_z] -> DisturbanceEstimationPhase2/11(intintFmenos_z), DisturbanceEstimationPhase1/14(intintFmenos_z)
  [GainRampDist3Value] -> DisturbanceEstimationPhase2/12(gain3), DisturbanceEstimationPhase1/15(gain3)
  [ExperimentTimeValue] -> MATLAB Sweep/5(EndTime)
  AmplitureRefSignalRead2/1 -> MATLAB Sweep/2(Amp)
  StartTimeSignalRead3/1 -> MATLAB Sweep/4(StartTime)
  SimTimeSignalRead4/1 -> MATLAB Sweep/1(Time)
  FreqRefSignalRead1/1 -> MATLAB Sweep/3(Freq)
  [DForce_Load] -> CommSystem/2(dFload)
  Constant2/1 -> Data Store Write14/1
  [Force_Load] -> CommSystem/1(Fload)
  [DPosEnc2] -> CommSystem/8(dX)
  [PosEnc2] -> CommSystem/7(X)
  [DForce_Hyd] -> CommSystem/4(dFhyd)
  [Pa] -> CommSystem/5(Pa)
  [Force_Hyd] -> CommSystem/3(Fhyd)
  [Pb] -> CommSystem/6(Pb)
  Divide1/1 -> Product11/1, [ControlAction]
  [Reference] -> CommSystem/9(Ref)
  [LastAction] -> CommSystem/10(last_action)
  [LastAction_RL] -> CommSystem/11(last_action_rl)
  [ControlAction] -> CommSystem/12(last_action_control)
  ADCReadToPressure3/1(y) -> Low-Pass Filter (Discrete or Continuous)8/1, Scope_Ptank/1
  ADC_CLASS1_BL3/1 -> ADCReadToPressure1/1(u)
  ForceHydOffset/1 -> Sum6/2
  Low-Pass Filter (Discrete or Continuous)2/1 -> PolyDerivativeSubSystem5/1(Signal), [PosEnc1], Scope_Pos1_Filter/1
  Gain2/1 -> Sum2/1
  Enc2StartPosition/1 -> Sum2/2
  Constant4/1 -> Cast To Boolean/1
  ADCReadToNewtons_Hyd/1(y) -> Gain1/1
  ADCReadToPressure/1(y) -> Scope_Pa/1, Low-Pass Filter (Discrete or Continuous)6/1
  ADC_CLASS1_BL1/1 -> ADCReadToNewtons_Hyd/1(u)
  ADC_CLASS1_BL4/1 -> ADCReadToNewtons_Load/1(u)
  Sum2/1 -> Product12/1, Low-Pass Filter (Discrete or Continuous)3/1, Scope_Pos2/1
  ADC_CLASS1_BL2/1 -> ADCReadToPressure/1(u)
  Sum6/1 -> Scope_Force_Hyd/1, Low-Pass Filter (Discrete or Continuous)7/1
  Gain/1 -> Gain2/1
  ForceLoadOffset/1 -> Sum7/2
  ADCReadToPressure1/1(y) -> Low-Pass Filter (Discrete or Continuous)5/1, Scope_Pb/1
  [PolyFitPoints] -> PolyDerivativeSubSystem1/2(N)
  [PolyFitPoints] -> PolyDerivativeSubSystem5/2(N)
  Low-Pass Filter (Discrete or Continuous)/1 -> PolyDerivativeSubSystem1/1(Signal), Discrete Derivative1/1, [Force_Load], Scope_Force_Load_Filter/1
  EMC_ENCODER_BL2/1 -> Gain/1
  [PolyFitPoints] -> PolyDerivativeSubSystem2/2(N)
  Sum7/1 -> Scope_Force_Load/1, Low-Pass Filter (Discrete or Continuous)/1
  Discrete Derivative1/1 -> Scope_DForce_Load_Old/1
  PolyDerivativeSubSystem2/1(dSignal) -> [DForce_Hyd], Scope_DForce_Hyd/1
  Low-Pass Filter (Discrete or Continuous)6/1 -> [Pa], Scope_Pa_Filter/1
  ADCReadToPressure2/1(y) -> Scope1/1, Low-Pass Filter (Discrete or Continuous)4/1, Scope_Psource/1
  ADCReadToNewtons_Load/1(y) -> Sum7/1
  Low-Pass Filter (Discrete or Continuous)3/1 -> Scope_Pos2_Filter/1, [PosEnc2], PolyDerivativeSubSystem3/1(Signal)
  ADC_CLASS1_BL6/1 -> ADCReadToPressure3/1(u)
  PolyDerivativeSubSystem3/2(ddSignal) -> [DDPosEnc2]
  Low-Pass Filter (Discrete or Continuous)5/1 -> [Pb], Scope_Pb_Filter/1
  Constant1/1 -> Product12/2
  Product12/1 -> Scope_SpringForce/1
  Low-Pass Filter (Discrete or Continuous)7/1 -> PolyDerivativeSubSystem2/1(Signal), [Force_Hyd], Scope_Force_Hyd_Filter/1
  PolyDerivativeSubSystem5/1(dSignal) -> [DPosEnc1]
  ADC_CLASS1_BL5/1 -> ADCReadToPressure2/1(u)
  Low-Pass Filter (Discrete or Continuous)4/1 -> [Psource], Scope_Psource_Filter/1
  EMC_ENCODER_BL1/1 -> Low-Pass Filter (Discrete or Continuous)2/1, Scope_Pos1/1
  Gain1/1 -> Sum6/1
  PolyDerivativeSubSystem1/1(dSignal) -> [DForce_Load], Scope_DForce_Load/1
  PolyDerivativeSubSystem3/1(dSignal) -> Scope5/1, [DPosEnc2]
  [PolyFitPoints] -> PolyDerivativeSubSystem3/2(N)
  Low-Pass Filter (Discrete or Continuous)8/1 -> Scope_Ptank_Filter/1, [Ptank]
  Cast To Boolean/1 -> ADC_CLASS1_BL6/1, ADC_CLASS1_BL5/1, ADC_CLASS1_BL1/1, ADC_CLASS1_BL2/1, ADC_CLASS1_BL3/1, ADC_CLASS1_BL4/1
  Constant5/1 -> [PolyFitPoints]
  MATLAB Function4/1(y) -> CommSystem/Enable
  Data Store Read31/1 -> ScopeCounter/1, MATLAB Function4/1(u1)
  Data Store Read33/1 -> MATLAB Function4/2(u2)
  MATLAB Function4/2(new_u1) -> Data Store Write15/1
  Data Store Read34/1 -> MATLAB Function4/3(u3), Edge Detector3/1
  Edge Detector3/1 -> MATLAB Function4/4(u4)
  RLgain/1 -> Product10/2
  RL_FL/1(y) -> RLAction/1, Product10/1
  ControlGain/1 -> Product11/2
  [g_HydModel] -> RL_FL/1(g)
  [ForceError] -> RL_FL/2(erro)
  [IntForceError] -> RL_FL/5(int_erro)
  Data Store Read35/1 -> [KpRl], ScopeKpRl/1, RL_FL/3(Kp)
  Data Store Read36/1 -> [KiRl], ScopeKiRl/1, RL_FL/4(Ki)
  Data Store Read37/1 -> RL_FL/6(flag_start)
  Product10/1 -> Saturation3/1
  Saturation3/1 -> Divide2/1
  [Un] -> Divide2/2
  Divide2/1 -> Sum5/2, [LastAction_RL]
  GradConst/1 -> [GradConst]
  DS1202SER_INT_C1_I1/1 -> Interrupt-Driven Reception/Trigger
  Product11/1 -> Sum5/1
  Switch1/1 -> Saturation6/1
  Data Store Read38/1 -> ScopeFlagStart/1, Switch1/2
  Data Store Read40/1 -> Discrete-Time Integrator4/2
  [Force_Load] -> Sum4/1
  Discrete-Time Integrator4/1 -> [IntPosError]
  Product13/1 -> Discrete-Time Integrator4/1
  Sum4/1 -> ScopeForceError1/1, Product13/1, PolyDerivativeSubSystem4/1(Signal), [PosError]
  Data Store Read39/1 -> Product13/2
  PolyDerivativeSubSystem4/1(dSignal) -> [DPosError]
  Data Store Read41/1 -> Product14/2
  Saturation4/1 -> Divide3/1
  [Un] -> Divide3/2
  Product14/1 -> Saturation4/1
  Product15/1 -> [PID_Value_Pos], ScopePID1/1
  [Kd_Pos] -> Product18/1
  Data Store Read9/1 -> Product15/2
  [IntPosError] -> Product17/2
  Sum8/1 -> Product15/1
  Product17/1 -> Sum8/1
  [Kp_Pos] -> Product16/2
  Product16/1 -> Sum8/2
  [PosError] -> Product16/1
  Product18/1 -> Sum8/3
  [Ki_Pos] -> Product17/1
  [DPosError] -> Product18/2
  FLcontroller1/1(y) -> Product14/1
  [f_HydMode] -> FLcontroller1/2(f)
  Data Store Read43/1 -> FLcontroller1/6(flag_start)
  [g_HydModel] -> FLcontroller1/3(g)
  Constant7/1 -> FLcontroller1/5(d), FLcontroller1/4(dFref)
  [PID_Value_Pos] -> FLcontroller1/1(pid)
  Kd_value1/1 -> [Kd_Pos]
  Ki_value1/1 -> [Ki_Pos]
  Kp_value1/1 -> [Kp_Pos]
  Divide3/1 -> Switch1/3
  Data Store Read44/1 -> Edge Detector4/1
  Edge Detector4/1 -> RefRand/1(flag)
  Data Store Read45/1 -> RefRand/2(amp)
  Data Store Read46/1 -> RefRand/3(freq)
  RefRand/1(new_amp) -> Data Store Write16/1
  RefRand/2(new_freq) -> Data Store Write17/1
  Saturation6/1 -> Gain3/1
  [Reference] -> ContractionMetricFilterSystem1/2(Ref)
  Mux/1 -> ContractionMetricFilterSystem1/1(state)
  [Force_Hyd] -> Mux/1
  [DForce_Hyd] -> Mux/2
  [Force_Load] -> Mux/3
  [DForce_Load] -> Mux/4
  [Pa] -> Mux/5
  [Pb] -> Mux/6
  [PosEnc2] -> Mux/7
  [DPosEnc2] -> Mux/8
  Data Store Read51/1 -> Product20/2
  ContractionMetricFilterSystem1/1(Current) -> Product20/1
  Product20/1 -> ScopeOutput/1, [LastAction], Data Store Write6/1, Switch1/1
  DiscreteContinousMode/1 -> [DiscreteContinousMode]
  SmoothFactor/1 -> [SmoothFactor]
  Random/1 -> RefRand/4(random)
  MaxFreq/1 -> RefRand/5(max_freq)
  Data Store Read32/1 -> Product/3
  Data Store Read47/1 -> RefRand/6(pos)
  RefRand/3(new_pos) -> Data Store Write18/1
  Data Store Read48/1 -> Sum4/2
  Product/1 -> MATLAB Function2/1(u)
  MATLAB Function2/1(y) -> Discrete Derivative3/1, ScopeRefSignal/1, [Reference]
  SimTimeSignalRead5/1 -> MATLAB Function2/3(time)
  StartTimeSignalRead4/1 -> MATLAB Function2/2(start)
  RefFunctionSin/2(new_amp) -> Data Store Write19/1
  controller_select/1 -> [ControllerSelect]
  start_freq/1 -> RefRand/7(start_freq)
  Cli/1 -> FunctionCalculateHydModel/21(cli)
  FunctionCalculateHydModel/5(leak) -> [leak]
